simulink model "myo_sfun_one_myo_imu_emg"  (R2019a)
(part 9 of 12)

  "IW{2,1}(917,:)'" : Constant  Value=[1.233818349995047913836287989397533237934112548828125;-1.4548391149698105540011283665080554783344268798828125;-0.57922557343483427327868184875114820897579193115234375;1.505800985853002149639223716803826391696929931640625;1.3314411941759825008801954027148894965648651123046875;0.383690991252394197896791183666209690272808074951171875;-1.31641986432559665587405106634832918643951416015625;-1.081150647899540739871326877619139850139617919921875]
      mask Display: e = 0.06;c1 = [120 150 230]/255;c2 = ([120 150 230]+0)/383;c3 = ([120 150 230]+128)/383;patch([0 1 1 0],[0 0 1 1],c1);patch([0 1 1 1-e 1-e 0+e],[0 0 1 1-e 0+e 0+e],c2);patch([0 0 1 1-e 0+e 0+e],[0 1 1 1-e 1-e 0+e],c3);plot([0 1 1 0 0],[0 0 1 1 0]);disp('weights');
  "IW{2,1}(918,:)'" : Constant  Value=[0.97625063577431225869673880879417993128299713134765625;-1.796096170135296432590621407143771648406982421875;-0.93306574008488973870356630868627689778804779052734375;0.3230690155631952276138463275856338441371917724609375;-1.6813590513011014149213906421209685504436492919921875;-0.0308654014504310715560908562338227056898176670074462890625;-1.698210746333440379629564631613902747631072998046875;-0.535703429127936114895192076801322400569915771484375]
      mask Display: e = 0.06;c1 = [120 150 230]/255;c2 = ([120 150 230]+0)/383;c3 = ([120 150 230]+128)/383;patch([0 1 1 0],[0 0 1 1],c1);patch([0 1 1 1-e 1-e 0+e],[0 0 1 1-e 0+e 0+e],c2);patch([0 0 1 1-e 0+e 0+e],[0 1 1 1-e 1-e 0+e],c3);plot([0 1 1 0 0],[0 0 1 1 0]);disp('weights');
  "IW{2,1}(919,:)'" : Constant  Value=[-0.062478952272413797175421024121533264406025409698486328125;-0.96688876038711268900982531704357825219631195068359375;-1.3113773268668922344915017674793489277362823486328125;1.2445006808411676058057082627783529460430145263671875;1.8892739940812457444252459026756696403026580810546875;0.91363180064540261415828581448295153677463531494140625;1.472319784430609512781984449247829616069793701171875;0.2367699596751023649598977272034971974790096282958984375]
      mask Display: e = 0.06;c1 = [120 150 230]/255;c2 = ([120 150 230]+0)/383;c3 = ([120 150 230]+128)/383;patch([0 1 1 0],[0 0 1 1],c1);patch([0 1 1 1-e 1-e 0+e],[0 0 1 1-e 0+e 0+e],c2);patch([0 0 1 1-e 0+e 0+e],[0 1 1 1-e 1-e 0+e],c3);plot([0 1 1 0 0],[0 0 1 1 0]);disp('weights');
  "IW{2,1}(92,:)'" : Constant  Value=[1.569622482339936286876991289318539202213287353515625;-1.6722158298112417273983965060324408113956451416015625;1.3747281294294364517583062479388900101184844970703125;-0.84787514995572943465873549939715303480625152587890625;0.7901565381123225595416670330450870096683502197265625;-0.508869894851785797840193481533788144588470458984375;-0.0235341566085378005313000215892316191457211971282958984375;1.5106950540518997438965698165702633559703826904296875]
      mask Display: e = 0.06;c1 = [120 150 230]/255;c2 = ([120 150 230]+0)/383;c3 = ([120 150 230]+128)/383;patch([0 1 1 0],[0 0 1 1],c1);patch([0 1 1 1-e 1-e 0+e],[0 0 1 1-e 0+e 0+e],c2);patch([0 0 1 1-e 0+e 0+e],[0 1 1 1-e 1-e 0+e],c3);plot([0 1 1 0 0],[0 0 1 1 0]);disp('weights');
  "IW{2,1}(920,:)'" : Constant  Value=[-1.78069224270060377790514394291676580905914306640625;-1.756790645973715481176213870639912784099578857421875;0.8717506085395985149233410993474535644054412841796875;0.632232144906200499434589801239781081676483154296875;0.09756681000700063999264699532432132400572299957275390625;1.5168287045180723904280739589012227952480316162109375;0.0183378640337535682436342909795712330378592014312744140625;-1.1205682288554947856340504586114548146724700927734375]
      mask Display: e = 0.06;c1 = [120 150 230]/255;c2 = ([120 150 230]+0)/383;c3 = ([120 150 230]+128)/383;patch([0 1 1 0],[0 0 1 1],c1);patch([0 1 1 1-e 1-e 0+e],[0 0 1 1-e 0+e 0+e],c2);patch([0 0 1 1-e 0+e 0+e],[0 1 1 1-e 1-e 0+e],c3);plot([0 1 1 0 0],[0 0 1 1 0]);disp('weights');
  "IW{2,1}(921,:)'" : Constant  Value=[1.2340381365703052551907603628933429718017578125;-0.7941917179881461397172870420035906136035919189453125;0.92869565930659325747598131783888675272464752197265625;-1.48036562469159260757578522316180169582366943359375;-1.2877727848034314916958464891649782657623291015625;1.4188258803790863016303092081216163933277130126953125;1.3505426288009514390608956091455183923244476318359375;0.56256213396588250486018978335778228938579559326171875]
      mask Display: e = 0.06;c1 = [120 150 230]/255;c2 = ([120 150 230]+0)/383;c3 = ([120 150 230]+128)/383;patch([0 1 1 0],[0 0 1 1],c1);patch([0 1 1 1-e 1-e 0+e],[0 0 1 1-e 0+e 0+e],c2);patch([0 0 1 1-e 0+e 0+e],[0 1 1 1-e 1-e 0+e],c3);plot([0 1 1 0 0],[0 0 1 1 0]);disp('weights');
  "IW{2,1}(922,:)'" : Constant  Value=[0.52907092398030197699654308962635695934295654296875;-0.56376371958651005922291687966207973659038543701171875;1.962985257292654051042291030171327292919158935546875;-1.296892178749799118264718345017172396183013916015625;0.4288987352076383263721481853281147778034210205078125;-1.2792060230482646954186520815710537135601043701171875;0.00643970491984885602676502713848094572313129901885986328125;-1.7085131522321892472149329478270374238491058349609375]
      mask Display: e = 0.06;c1 = [120 150 230]/255;c2 = ([120 150 230]+0)/383;c3 = ([120 150 230]+128)/383;patch([0 1 1 0],[0 0 1 1],c1);patch([0 1 1 1-e 1-e 0+e],[0 0 1 1-e 0+e 0+e],c2);patch([0 0 1 1-e 0+e 0+e],[0 1 1 1-e 1-e 0+e],c3);plot([0 1 1 0 0],[0 0 1 1 0]);disp('weights');
  "IW{2,1}(923,:)'" : Constant  Value=[-1.4344793229196290962335069707478396594524383544921875;-1.433847325507824788104471736005507409572601318359375;0.85757048812909852930630449918680824339389801025390625;1.4320646508188261680771802275558002293109893798828125;0.7544209783935496016482602499308995902538299560546875;0.60201451337752731607366740718134678900241851806640625;-1.0747759747253453621596008815686218440532684326171875;-1.4299949869762149656793326357728801667690277099609375]
      mask Display: e = 0.06;c1 = [120 150 230]/255;c2 = ([120 150 230]+0)/383;c3 = ([120 150 230]+128)/383;patch([0 1 1 0],[0 0 1 1],c1);patch([0 1 1 1-e 1-e 0+e],[0 0 1 1-e 0+e 0+e],c2);patch([0 0 1 1-e 0+e 0+e],[0 1 1 1-e 1-e 0+e],c3);plot([0 1 1 0 0],[0 0 1 1 0]);disp('weights');
  "IW{2,1}(924,:)'" : Constant  Value=[1.46370152051110746782569549395702779293060302734375;-1.45028040887480802467734974925406277179718017578125;-1.693963962550077528845804408774711191654205322265625;-1.3273955542829203313459629498538561165332794189453125;0.2477303836859091890065798224895843304693698883056640625;0.410986296970826614494143314004759304225444793701171875;-1.34217386380958725311529633472673594951629638671875;0.334924337123925497383680749408085830509662628173828125]
      mask Display: e = 0.06;c1 = [120 150 230]/255;c2 = ([120 150 230]+0)/383;c3 = ([120 150 230]+128)/383;patch([0 1 1 0],[0 0 1 1],c1);patch([0 1 1 1-e 1-e 0+e],[0 0 1 1-e 0+e 0+e],c2);patch([0 0 1 1-e 0+e 0+e],[0 1 1 1-e 1-e 0+e],c3);plot([0 1 1 0 0],[0 0 1 1 0]);disp('weights');
  "IW{2,1}(925,:)'" : Constant  Value=[-0.80343815628262149619587262350250966846942901611328125;1.23324691550459508704307154403068125247955322265625;-0.316568060198488876455513718610745854675769805908203125;-1.945293161466664866310338766197673976421356201171875;0.5960065168583223993437059107236564159393310546875;1.6328048241174808463682666115346364676952362060546875;-1.23835047078790072561105262138880789279937744140625;-0.65057393111039230060299587421468459069728851318359375]
      mask Display: e = 0.06;c1 = [120 150 230]/255;c2 = ([120 150 230]+0)/383;c3 = ([120 150 230]+128)/383;patch([0 1 1 0],[0 0 1 1],c1);patch([0 1 1 1-e 1-e 0+e],[0 0 1 1-e 0+e 0+e],c2);patch([0 0 1 1-e 0+e 0+e],[0 1 1 1-e 1-e 0+e],c3);plot([0 1 1 0 0],[0 0 1 1 0]);disp('weights');
  "IW{2,1}(926,:)'" : Constant  Value=[0.09118175811866091606816553394310176372528076171875;-0.8389622353409638133570069840061478316783905029296875;1.210727032626933041825623149634338915348052978515625;1.293501909600718757786808055243454873561859130859375;-1.6284239784387757321582057556952349841594696044921875;-1.60098607932530256903191911987960338592529296875;-1.2636191412525807908906472221133299171924591064453125;-0.36179817522204160695764585398137569427490234375]
      mask Display: e = 0.06;c1 = [120 150 230]/255;c2 = ([120 150 230]+0)/383;c3 = ([120 150 230]+128)/383;patch([0 1 1 0],[0 0 1 1],c1);patch([0 1 1 1-e 1-e 0+e],[0 0 1 1-e 0+e 0+e],c2);patch([0 0 1 1-e 0+e 0+e],[0 1 1 1-e 1-e 0+e],c3);plot([0 1 1 0 0],[0 0 1 1 0]);disp('weights');
  "IW{2,1}(927,:)'" : Constant  Value=[-1.4683117468887691980938825508928857743740081787109375;-1.125812298427818713975057107745669782161712646484375;1.402350909702253289879081421531736850738525390625;1.17972039460394029219969525001943111419677734375;-1.189874093891304607240044788341037929058074951171875;0.82527880489423888210609447924070991575717926025390625;1.3554320717921399808147953081061132252216339111328125;0.445007997019099266200470310650416649878025054931640625]
      mask Display: e = 0.06;c1 = [120 150 230]/255;c2 = ([120 150 230]+0)/383;c3 = ([120 150 230]+128)/383;patch([0 1 1 0],[0 0 1 1],c1);patch([0 1 1 1-e 1-e 0+e],[0 0 1 1-e 0+e 0+e],c2);patch([0 0 1 1-e 0+e 0+e],[0 1 1 1-e 1-e 0+e],c3);plot([0 1 1 0 0],[0 0 1 1 0]);disp('weights');
  "IW{2,1}(928,:)'" : Constant  Value=[0.20559520258321006824786536526517011225223541259765625;0.3496458011807741517174008549773134291172027587890625;0.7578976435515378806684338997001759707927703857421875;-0.96497414503002676422482863927143625915050506591796875;-2.2761285455608035732666394324041903018951416015625;-2.114827771400021649839118254021741449832916259765625;0.5069606864833466897124480965430848300457000732421875;0.53269535080165086871062385398545302450656890869140625]
      mask Display: e = 0.06;c1 = [120 150 230]/255;c2 = ([120 150 230]+0)/383;c3 = ([120 150 230]+128)/383;patch([0 1 1 0],[0 0 1 1],c1);patch([0 1 1 1-e 1-e 0+e],[0 0 1 1-e 0+e 0+e],c2);patch([0 0 1 1-e 0+e 0+e],[0 1 1 1-e 1-e 0+e],c3);plot([0 1 1 0 0],[0 0 1 1 0]);disp('weights');
  "IW{2,1}(929,:)'" : Constant  Value=[0.83300144991458946464035761891864240169525146484375;-1.0378524650019234076836482927319593727588653564453125;-0.1574880296440317462014490956789813935756683349609375;-0.158074214384277933476141697610728442668914794921875;1.3647263842503016828544559757574461400508880615234375;1.2931349855028388962097096737124957144260406494140625;-0.040154367939153355615555796020998968742787837982177734375;2.380261894743207928826222996576689183712005615234375]
      mask Display: e = 0.06;c1 = [120 150 230]/255;c2 = ([120 150 230]+0)/383;c3 = ([120 150 230]+128)/383;patch([0 1 1 0],[0 0 1 1],c1);patch([0 1 1 1-e 1-e 0+e],[0 0 1 1-e 0+e 0+e],c2);patch([0 0 1 1-e 0+e 0+e],[0 1 1 1-e 1-e 0+e],c3);plot([0 1 1 0 0],[0 0 1 1 0]);disp('weights');
  "IW{2,1}(93,:)'" : Constant  Value=[-1.251296272410225896010160795412957668304443359375;1.501077551730921388895012569264508783817291259765625;-1.20650068227487228256222806521691381931304931640625;-1.4767900871354211478347906449926085770130157470703125;1.23206725601141098280777441686950623989105224609375;0.6159584242327740266631508347927592694759368896484375;-0.61376517944694908290870216660550795495510101318359375;1.160008933468915426345802188734523952007293701171875]
      mask Display: e = 0.06;c1 = [120 150 230]/255;c2 = ([120 150 230]+0)/383;c3 = ([120 150 230]+128)/383;patch([0 1 1 0],[0 0 1 1],c1);patch([0 1 1 1-e 1-e 0+e],[0 0 1 1-e 0+e 0+e],c2);patch([0 0 1 1-e 0+e 0+e],[0 1 1 1-e 1-e 0+e],c3);plot([0 1 1 0 0],[0 0 1 1 0]);disp('weights');
  "IW{2,1}(930,:)'" : Constant  Value=[0.459515014521598208485642089726752601563930511474609375;1.274038251996577830738033298985101282596588134765625;-0.462123489601668213655472072787233628332614898681640625;-1.2313600730026921237225678851245902478694915771484375;2.324661295404313765544657144346274435520172119140625;-1.275147702745309974403653541230596601963043212890625;0.006852607156798958508436836467581088072620332241058349609375;0.64580748349911776262644025337067432701587677001953125]
      mask Display: e = 0.06;c1 = [120 150 230]/255;c2 = ([120 150 230]+0)/383;c3 = ([120 150 230]+128)/383;patch([0 1 1 0],[0 0 1 1],c1);patch([0 1 1 1-e 1-e 0+e],[0 0 1 1-e 0+e 0+e],c2);patch([0 0 1 1-e 0+e 0+e],[0 1 1 1-e 1-e 0+e],c3);plot([0 1 1 0 0],[0 0 1 1 0]);disp('weights');
  "IW{2,1}(931,:)'" : Constant  Value=[0.1280454771649393863608423771438538096845149993896484375;0.59353344051585155138894833726226352155208587646484375;-1.2413483482938836299780405170167796313762664794921875;-1.387491740431027853475143274408765137195587158203125;-0.41476915329622709993628859592718072235584259033203125;2.049464981171696731365727828233502805233001708984375;0.94176951285771381972011795369326137006282806396484375;-1.3840451161403819480000265684793703258037567138671875]
      mask Display: e = 0.06;c1 = [120 150 230]/255;c2 = ([120 150 230]+0)/383;c3 = ([120 150 230]+128)/383;patch([0 1 1 0],[0 0 1 1],c1);patch([0 1 1 1-e 1-e 0+e],[0 0 1 1-e 0+e 0+e],c2);patch([0 0 1 1-e 0+e 0+e],[0 1 1 1-e 1-e 0+e],c3);plot([0 1 1 0 0],[0 0 1 1 0]);disp('weights');
  "IW{2,1}(932,:)'" : Constant  Value=[0.35977187717559921953380808190559037029743194580078125;1.7540295201390023738241552564431913197040557861328125;-1.43762591560315744487752454006113111972808837890625;-0.006080287386095576708522347786356476717628538608551025390625;-0.311097464246324062475679284034413285553455352783203125;-1.2697604847810930461804446167661808431148529052734375;0.94609842053890746971234193551936186850070953369140625;1.77723577742588734196260702447034418582916259765625]
      mask Display: e = 0.06;c1 = [120 150 230]/255;c2 = ([120 150 230]+0)/383;c3 = ([120 150 230]+128)/383;patch([0 1 1 0],[0 0 1 1],c1);patch([0 1 1 1-e 1-e 0+e],[0 0 1 1-e 0+e 0+e],c2);patch([0 0 1 1-e 0+e 0+e],[0 1 1 1-e 1-e 0+e],c3);plot([0 1 1 0 0],[0 0 1 1 0]);disp('weights');
  "IW{2,1}(933,:)'" : Constant  Value=[-0.55971507988235524866382775144302286207675933837890625;1.344039743685524701533040570211596786975860595703125;1.284763347918191467300630392855964601039886474609375;-1.55473640286817182953882365836761891841888427734375;-1.488883701200015341470361818210221827030181884765625;-0.14626156873139828373808768446906469762325286865234375;-0.6249568527413627005984153583995066583156585693359375;-1.4858424850743496836713575248722918331623077392578125]
      mask Display: e = 0.06;c1 = [120 150 230]/255;c2 = ([120 150 230]+0)/383;c3 = ([120 150 230]+128)/383;patch([0 1 1 0],[0 0 1 1],c1);patch([0 1 1 1-e 1-e 0+e],[0 0 1 1-e 0+e 0+e],c2);patch([0 0 1 1-e 0+e 0+e],[0 1 1 1-e 1-e 0+e],c3);plot([0 1 1 0 0],[0 0 1 1 0]);disp('weights');
  "IW{2,1}(934,:)'" : Constant  Value=[-1.752013618542566320002151769585907459259033203125;1.3291169268141735937405201184446923434734344482421875;-0.6787032919514575102226672242977656424045562744140625;0.490359468964445321947920319871627725660800933837890625;-1.57210680514284195652408016030676662921905517578125;-0.01000360648531075681566537838307340280152857303619384765625;-0.285459327197532142239566610442125238478183746337890625;-1.7110715408113696955894056372926570475101470947265625]
      mask Display: e = 0.06;c1 = [120 150 230]/255;c2 = ([120 150 230]+0)/383;c3 = ([120 150 230]+128)/383;patch([0 1 1 0],[0 0 1 1],c1);patch([0 1 1 1-e 1-e 0+e],[0 0 1 1-e 0+e 0+e],c2);patch([0 0 1 1-e 0+e 0+e],[0 1 1 1-e 1-e 0+e],c3);plot([0 1 1 0 0],[0 0 1 1 0]);disp('weights');
  "IW{2,1}(935,:)'" : Constant  Value=[-1.6614565255023199252804033676511608064174652099609375;0.734584289137682588943789596669375896453857421875;1.0579080812622836393899206086643971502780914306640625;0.52610990226821907622678509142133407294750213623046875;1.34837736401491969928656544652767479419708251953125;1.0300380949842151689921365687041543424129486083984375;-0.87449305309208369418882966783712618052959442138671875;1.5773892164364966550493818431277759373188018798828125]
      mask Display: e = 0.06;c1 = [120 150 230]/255;c2 = ([120 150 230]+0)/383;c3 = ([120 150 230]+128)/383;patch([0 1 1 0],[0 0 1 1],c1);patch([0 1 1 1-e 1-e 0+e],[0 0 1 1-e 0+e 0+e],c2);patch([0 0 1 1-e 0+e 0+e],[0 1 1 1-e 1-e 0+e],c3);plot([0 1 1 0 0],[0 0 1 1 0]);disp('weights');
  "IW{2,1}(936,:)'" : Constant  Value=[0.022714479700087643332384601535522961057722568511962890625;-1.573558474179254318414677982218563556671142578125;1.3066200625597179652004342642612755298614501953125;-0.1673441857289472423087062225022236816585063934326171875;1.8960528148548283500218758490518666803836822509765625;1.340663180394818798646383584127761423587799072265625;0.55978272292861486203463527999701909720897674560546875;1.049900791636255714678327422006987035274505615234375]
      mask Display: e = 0.06;c1 = [120 150 230]/255;c2 = ([120 150 230]+0)/383;c3 = ([120 150 230]+128)/383;patch([0 1 1 0],[0 0 1 1],c1);patch([0 1 1 1-e 1-e 0+e],[0 0 1 1-e 0+e 0+e],c2);patch([0 0 1 1-e 0+e 0+e],[0 1 1 1-e 1-e 0+e],c3);plot([0 1 1 0 0],[0 0 1 1 0]);disp('weights');
  "IW{2,1}(937,:)'" : Constant  Value=[0.829643574270976902340635206201113760471343994140625;2.22733223083989262391924057737924158573150634765625;-0.79551413202837040206105712059070356190204620361328125;0.9418309463257037439376517795608378946781158447265625;-0.774473438339178255063188771600835025310516357421875;1.300848255993976909650200468604452908039093017578125;1.2493782215186015616126269378582946956157684326171875;0.021557995414638909947857570159612805582582950592041015625]
      mask Display: e = 0.06;c1 = [120 150 230]/255;c2 = ([120 150 230]+0)/383;c3 = ([120 150 230]+128)/383;patch([0 1 1 0],[0 0 1 1],c1);patch([0 1 1 1-e 1-e 0+e],[0 0 1 1-e 0+e 0+e],c2);patch([0 0 1 1-e 0+e 0+e],[0 1 1 1-e 1-e 0+e],c3);plot([0 1 1 0 0],[0 0 1 1 0]);disp('weights');
  "IW{2,1}(938,:)'" : Constant  Value=[1.345901355534946386427463949075900018215179443359375;-2.02660768801359747470769434585236012935638427734375;1.352468657955171682516493092407472431659698486328125;-1.3978356390675228393405404858640395104885101318359375;-0.9061008277153874690412749259849078953266143798828125;-0.0980897452544215731062848817600752227008342742919921875;0.72250261894200551449074509946512989699840545654296875;-0.209980731838069145656078262618393637239933013916015625]
      mask Display: e = 0.06;c1 = [120 150 230]/255;c2 = ([120 150 230]+0)/383;c3 = ([120 150 230]+128)/383;patch([0 1 1 0],[0 0 1 1],c1);patch([0 1 1 1-e 1-e 0+e],[0 0 1 1-e 0+e 0+e],c2);patch([0 0 1 1-e 0+e 0+e],[0 1 1 1-e 1-e 0+e],c3);plot([0 1 1 0 0],[0 0 1 1 0]);disp('weights');
  "IW{2,1}(939,:)'" : Constant  Value=[-0.82112012880838258777060900683864019811153411865234375;-1.930845595022031790932715011877007782459259033203125;-1.15556707295993010831125502591021358966827392578125;1.179015320370934372107285525999031960964202880859375;-1.3288541314620074818009243244887329638004302978515625;1.2953923768230557467262542559183202683925628662109375;-0.2042937924653980275024878210388123989105224609375;-0.6321215672831559384547972513246349990367889404296875]
      mask Display: e = 0.06;c1 = [120 150 230]/255;c2 = ([120 150 230]+0)/383;c3 = ([120 150 230]+128)/383;patch([0 1 1 0],[0 0 1 1],c1);patch([0 1 1 1-e 1-e 0+e],[0 0 1 1-e 0+e 0+e],c2);patch([0 0 1 1-e 0+e 0+e],[0 1 1 1-e 1-e 0+e],c3);plot([0 1 1 0 0],[0 0 1 1 0]);disp('weights');
  "IW{2,1}(94,:)'" : Constant  Value=[-0.89691044877446557403999349844525568187236785888671875;-1.9703867433167996381371267489157617092132568359375;-1.2689724396955994745184170824359171092510223388671875;-1.102188217761382649229062735685147345066070556640625;0.212948896185985281359620557850576005876064300537109375;1.4063245905018693093779802438803017139434814453125;0.5220856679645944353751474409364163875579833984375;1.2669379614301450320823505535372532904148101806640625]
      mask Display: e = 0.06;c1 = [120 150 230]/255;c2 = ([120 150 230]+0)/383;c3 = ([120 150 230]+128)/383;patch([0 1 1 0],[0 0 1 1],c1);patch([0 1 1 1-e 1-e 0+e],[0 0 1 1-e 0+e 0+e],c2);patch([0 0 1 1-e 0+e 0+e],[0 1 1 1-e 1-e 0+e],c3);plot([0 1 1 0 0],[0 0 1 1 0]);disp('weights');
  "IW{2,1}(940,:)'" : Constant  Value=[-1.9284641361261212200162162844208069145679473876953125;-0.6923000284259206438264300231821835041046142578125;-0.01547752074768899387124942990112685947678983211517333984375;-1.51835172518999694801777877728454768657684326171875;1.1196957434104588546830427731038071215152740478515625;-0.54044636995000117085652391324401833117008209228515625;-0.40395263561673733221368820522911846637725830078125;-1.6755700378273326034417323171510361135005950927734375]
      mask Display: e = 0.06;c1 = [120 150 230]/255;c2 = ([120 150 230]+0)/383;c3 = ([120 150 230]+128)/383;patch([0 1 1 0],[0 0 1 1],c1);patch([0 1 1 1-e 1-e 0+e],[0 0 1 1-e 0+e 0+e],c2);patch([0 0 1 1-e 0+e 0+e],[0 1 1 1-e 1-e 0+e],c3);plot([0 1 1 0 0],[0 0 1 1 0]);disp('weights');
  "IW{2,1}(941,:)'" : Constant  Value=[-0.67344134392942589517616625016671605408191680908203125;-1.7808742618691166814670623352867551147937774658203125;1.4264091809267844812580960933701135218143463134765625;1.911975433919925304593334658420644700527191162109375;-0.7236950162813198250688628831994719803333282470703125;-0.370798693591568639948974350772914476692676544189453125;-0.329395901859115713961045912583358585834503173828125;-0.96579283248583458476588248231564648449420928955078125]
      mask Display: e = 0.06;c1 = [120 150 230]/255;c2 = ([120 150 230]+0)/383;c3 = ([120 150 230]+128)/383;patch([0 1 1 0],[0 0 1 1],c1);patch([0 1 1 1-e 1-e 0+e],[0 0 1 1-e 0+e 0+e],c2);patch([0 0 1 1-e 0+e 0+e],[0 1 1 1-e 1-e 0+e],c3);plot([0 1 1 0 0],[0 0 1 1 0]);disp('weights');
  "IW{2,1}(942,:)'" : Constant  Value=[-1.64674280850280663202056530280970036983489990234375;-1.5001296336770109096647729529649950563907623291015625;0.08935031672762583365710042926366440951824188232421875;-0.921153845618884137280701907002367079257965087890625;-0.483100667039175146744156563727301545441150665283203125;-0.7427427715172323363646000871085561811923980712890625;-1.6797167079109793785818283140542916953563690185546875;-1.26337657129443758918796447687782347202301025390625]
      mask Display: e = 0.06;c1 = [120 150 230]/255;c2 = ([120 150 230]+0)/383;c3 = ([120 150 230]+128)/383;patch([0 1 1 0],[0 0 1 1],c1);patch([0 1 1 1-e 1-e 0+e],[0 0 1 1-e 0+e 0+e],c2);patch([0 0 1 1-e 0+e 0+e],[0 1 1 1-e 1-e 0+e],c3);plot([0 1 1 0 0],[0 0 1 1 0]);disp('weights');
  "IW{2,1}(943,:)'" : Constant  Value=[-0.6229731159529052764156631383229978382587432861328125;0.98169370896949093019401288984226994216442108154296875;-1.6364243634393706994245576424873434007167816162109375;0.950796335976273443435502485954202711582183837890625;1.0949390867111337133366077978280372917652130126953125;1.515828966336887351218365438398905098438262939453125;0.9413789297321477622659813278005458414554595947265625;-1.229582187669542303609659938956610858440399169921875]
      mask Display: e = 0.06;c1 = [120 150 230]/255;c2 = ([120 150 230]+0)/383;c3 = ([120 150 230]+128)/383;patch([0 1 1 0],[0 0 1 1],c1);patch([0 1 1 1-e 1-e 0+e],[0 0 1 1-e 0+e 0+e],c2);patch([0 0 1 1-e 0+e 0+e],[0 1 1 1-e 1-e 0+e],c3);plot([0 1 1 0 0],[0 0 1 1 0]);disp('weights');
  "IW{2,1}(944,:)'" : Constant  Value=[1.6916018903944003426431663683615624904632568359375;1.630736797217114286695505143143236637115478515625;1.2800499861010774527159128410858102142810821533203125;0.94571459497293342000290294890874065458774566650390625;0.3303592853984034238834510688320733606815338134765625;-1.4924581285519600282185592732275836169719696044921875;-0.79231501501053436253840800418402068316936492919921875;-0.03770714380415697564163934885073103941977024078369140625]
      mask Display: e = 0.06;c1 = [120 150 230]/255;c2 = ([120 150 230]+0)/383;c3 = ([120 150 230]+128)/383;patch([0 1 1 0],[0 0 1 1],c1);patch([0 1 1 1-e 1-e 0+e],[0 0 1 1-e 0+e 0+e],c2);patch([0 0 1 1-e 0+e 0+e],[0 1 1 1-e 1-e 0+e],c3);plot([0 1 1 0 0],[0 0 1 1 0]);disp('weights');
  "IW{2,1}(945,:)'" : Constant  Value=[-0.07490041787247413151984432033714256249368190765380859375;-0.2172170720689318990093141792385722510516643524169921875;0.75781279649731825287517494871281087398529052734375;1.821447104661903182432070025242865085601806640625;-0.7881694043895723922332763322629034519195556640625;-1.684895341352864672757050357176922261714935302734375;-0.2646422506319991985179740368039347231388092041015625;-1.8832174078616155110665886240894906222820281982421875]
      mask Display: e = 0.06;c1 = [120 150 230]/255;c2 = ([120 150 230]+0)/383;c3 = ([120 150 230]+128)/383;patch([0 1 1 0],[0 0 1 1],c1);patch([0 1 1 1-e 1-e 0+e],[0 0 1 1-e 0+e 0+e],c2);patch([0 0 1 1-e 0+e 0+e],[0 1 1 1-e 1-e 0+e],c3);plot([0 1 1 0 0],[0 0 1 1 0]);disp('weights');
  "IW{2,1}(946,:)'" : Constant  Value=[-1.61656003434635398008367701550014317035675048828125;-1.5618385803786349885768913736683316528797149658203125;-0.277455301741910964619108881379361264407634735107421875;1.3992954332120628446745058681699447333812713623046875;-1.3023534400012752865194443074869923293590545654296875;0.9148572075036749406962144348653964698314666748046875;0.247215396692398059474982119354535825550556182861328125;-1.1568899404959995802499861383694224059581756591796875]
      mask Display: e = 0.06;c1 = [120 150 230]/255;c2 = ([120 150 230]+0)/383;c3 = ([120 150 230]+128)/383;patch([0 1 1 0],[0 0 1 1],c1);patch([0 1 1 1-e 1-e 0+e],[0 0 1 1-e 0+e 0+e],c2);patch([0 0 1 1-e 0+e 0+e],[0 1 1 1-e 1-e 0+e],c3);plot([0 1 1 0 0],[0 0 1 1 0]);disp('weights');
  "IW{2,1}(947,:)'" : Constant  Value=[0.67278616972188653999609186939778737723827362060546875;0.315790583508263000833693467939156107604503631591796875;-1.9304221908873084867508396200719289481639862060546875;1.46464184402568076137640673550777137279510498046875;0.324555519664747660346648672202718444168567657470703125;1.8096189180068671387147105633630417287349700927734375;-0.297396691982909022744507865354535169899463653564453125;-1.06090862285816722732079142588190734386444091796875]
      mask Display: e = 0.06;c1 = [120 150 230]/255;c2 = ([120 150 230]+0)/383;c3 = ([120 150 230]+128)/383;patch([0 1 1 0],[0 0 1 1],c1);patch([0 1 1 1-e 1-e 0+e],[0 0 1 1-e 0+e 0+e],c2);patch([0 0 1 1-e 0+e 0+e],[0 1 1 1-e 1-e 0+e],c3);plot([0 1 1 0 0],[0 0 1 1 0]);disp('weights');
  "IW{2,1}(948,:)'" : Constant  Value=[0.69274726211865711444914950334350578486919403076171875;1.75931371522753021707785592298023402690887451171875;-0.334146673453465548053742395495646633207798004150390625;1.416235474757840062665081859449855983257293701171875;-1.49001771332762444899344700388610363006591796875;-0.4963658635882872705025192772154696285724639892578125;1.6882243163268089158890461476403288543224334716796875;-0.106785619132828191180095700474339537322521209716796875]
      mask Display: e = 0.06;c1 = [120 150 230]/255;c2 = ([120 150 230]+0)/383;c3 = ([120 150 230]+128)/383;patch([0 1 1 0],[0 0 1 1],c1);patch([0 1 1 1-e 1-e 0+e],[0 0 1 1-e 0+e 0+e],c2);patch([0 0 1 1-e 0+e 0+e],[0 1 1 1-e 1-e 0+e],c3);plot([0 1 1 0 0],[0 0 1 1 0]);disp('weights');
  "IW{2,1}(949,:)'" : Constant  Value=[0.26027926239215359860423859572620131075382232666015625;0.55307858353162020481619265410699881613254547119140625;1.051142655215786536615496515878476202487945556640625;-1.3810340222430579348866785949212498962879180908203125;1.3515319635994840208326195352128706872463226318359375;1.838861764011227695192474129726178944110870361328125;-1.0853865001339315643491545415599830448627471923828125;1.115992553842682699638544363551773130893707275390625]
      mask Display: e = 0.06;c1 = [120 150 230]/255;c2 = ([120 150 230]+0)/383;c3 = ([120 150 230]+128)/383;patch([0 1 1 0],[0 0 1 1],c1);patch([0 1 1 1-e 1-e 0+e],[0 0 1 1-e 0+e 0+e],c2);patch([0 0 1 1-e 0+e 0+e],[0 1 1 1-e 1-e 0+e],c3);plot([0 1 1 0 0],[0 0 1 1 0]);disp('weights');
  "IW{2,1}(95,:)'" : Constant  Value=[0.005290517661980498852203336213051443337462842464447021484375;-1.6497505516666877145581793229212053120136260986328125;1.620443822731480576493368062074296176433563232421875;0.16986718877335504895853546258877031505107879638671875;1.054192073111287708542249674792401492595672607421875;2.0288246145218096216922276653349399566650390625;0.76925751328801295070292098898789845407009124755859375;0.305950453478517570005124071030877530574798583984375]
      mask Display: e = 0.06;c1 = [120 150 230]/255;c2 = ([120 150 230]+0)/383;c3 = ([120 150 230]+128)/383;patch([0 1 1 0],[0 0 1 1],c1);patch([0 1 1 1-e 1-e 0+e],[0 0 1 1-e 0+e 0+e],c2);patch([0 0 1 1-e 0+e 0+e],[0 1 1 1-e 1-e 0+e],c3);plot([0 1 1 0 0],[0 0 1 1 0]);disp('weights');
  "IW{2,1}(950,:)'" : Constant  Value=[0.2118013824636972020076797207366325892508029937744140625;0.0222517894993314417628749168898139032535254955291748046875;-0.59674814348700089272625746161793358623981475830078125;0.11734950071789367054275743385005625896155834197998046875;-1.024961618939134400108059708145447075366973876953125;1.9878634122041984877427012179396115243434906005859375;0.2500324382013621171694239819771610200405120849609375;2.353073982785186313293479543062858283519744873046875]
      mask Display: e = 0.06;c1 = [120 150 230]/255;c2 = ([120 150 230]+0)/383;c3 = ([120 150 230]+128)/383;patch([0 1 1 0],[0 0 1 1],c1);patch([0 1 1 1-e 1-e 0+e],[0 0 1 1-e 0+e 0+e],c2);patch([0 0 1 1-e 0+e 0+e],[0 1 1 1-e 1-e 0+e],c3);plot([0 1 1 0 0],[0 0 1 1 0]);disp('weights');
  "IW{2,1}(951,:)'" : Constant  Value=[-0.80119265775817571917372106327093206346035003662109375;0.29490648552127052273164053985965438187122344970703125;1.9174919947240212092509636931936256587505340576171875;2.132198923601664741767081068246625363826751708984375;0.60462532016717485117140995498630218207836151123046875;0.819228102816961012422325438819825649261474609375;-1.0039939427206672206693838234059512615203857421875;0.252263222953873877951735948954592458903789520263671875]
      mask Display: e = 0.06;c1 = [120 150 230]/255;c2 = ([120 150 230]+0)/383;c3 = ([120 150 230]+128)/383;patch([0 1 1 0],[0 0 1 1],c1);patch([0 1 1 1-e 1-e 0+e],[0 0 1 1-e 0+e 0+e],c2);patch([0 0 1 1-e 0+e 0+e],[0 1 1 1-e 1-e 0+e],c3);plot([0 1 1 0 0],[0 0 1 1 0]);disp('weights');
  "IW{2,1}(952,:)'" : Constant  Value=[-1.11396737416281599308831573580391705036163330078125;-1.3865399781131342304973941281787119805812835693359375;-0.40695912110590881649585526247392408549785614013671875;1.5312662831779870753479144696029834449291229248046875;-1.49056243641590224768833650159649550914764404296875;-0.97778759670928161451541882343008182942867279052734375;1.459003140404683929176599122001789510250091552734375;0.1557717566069929671090932288279873318970203399658203125]
      mask Display: e = 0.06;c1 = [120 150 230]/255;c2 = ([120 150 230]+0)/383;c3 = ([120 150 230]+128)/383;patch([0 1 1 0],[0 0 1 1],c1);patch([0 1 1 1-e 1-e 0+e],[0 0 1 1-e 0+e 0+e],c2);patch([0 0 1 1-e 0+e 0+e],[0 1 1 1-e 1-e 0+e],c3);plot([0 1 1 0 0],[0 0 1 1 0]);disp('weights');
  "IW{2,1}(953,:)'" : Constant  Value=[0.258251700948573026384025297375046648085117340087890625;-0.67611337492076251098893635571585036814212799072265625;-1.603811521270914308701094341813586652278900146484375;-0.5681734588386808670890104622230865061283111572265625;1.8536189902244133431707950876443646848201751708984375;-1.97368043547795668501976251718588173389434814453125;-0.5127002050856710457793496971135027706623077392578125;-0.414385209771393092648139599987189285457134246826171875]
      mask Display: e = 0.06;c1 = [120 150 230]/255;c2 = ([120 150 230]+0)/383;c3 = ([120 150 230]+128)/383;patch([0 1 1 0],[0 0 1 1],c1);patch([0 1 1 1-e 1-e 0+e],[0 0 1 1-e 0+e 0+e],c2);patch([0 0 1 1-e 0+e 0+e],[0 1 1 1-e 1-e 0+e],c3);plot([0 1 1 0 0],[0 0 1 1 0]);disp('weights');
  "IW{2,1}(954,:)'" : Constant  Value=[-0.0714688518537866246393974734019138850271701812744140625;0.18673843709045756522613146444200538098812103271484375;-0.9915786198777654103508893967955373227596282958984375;-1.5692759919708876292787635975400917232036590576171875;1.3352769605693486365538547033793292939662933349609375;1.4898625418610567106014741511899046599864959716796875;1.77523436073847307170581188984215259552001953125;-0.30240620026603981518320551913348026573657989501953125]
      mask Display: e = 0.06;c1 = [120 150 230]/255;c2 = ([120 150 230]+0)/383;c3 = ([120 150 230]+128)/383;patch([0 1 1 0],[0 0 1 1],c1);patch([0 1 1 1-e 1-e 0+e],[0 0 1 1-e 0+e 0+e],c2);patch([0 0 1 1-e 0+e 0+e],[0 1 1 1-e 1-e 0+e],c3);plot([0 1 1 0 0],[0 0 1 1 0]);disp('weights');
  "IW{2,1}(955,:)'" : Constant  Value=[-1.0269687330708421324487744641373865306377410888671875;-1.0798366757184023612126111402176320552825927734375;-0.69043258483427205618454536306671798229217529296875;-0.1303232596325844816487204980148817412555217742919921875;-1.93219267415173590052290819585323333740234375;-1.670762241355885802107650306425057351589202880859375;-1.102255017013542559567440548562444746494293212890625;-0.7532878530168323205629121730453334748744964599609375]
      mask Display: e = 0.06;c1 = [120 150 230]/255;c2 = ([120 150 230]+0)/383;c3 = ([120 150 230]+128)/383;patch([0 1 1 0],[0 0 1 1],c1);patch([0 1 1 1-e 1-e 0+e],[0 0 1 1-e 0+e 0+e],c2);patch([0 0 1 1-e 0+e 0+e],[0 1 1 1-e 1-e 0+e],c3);plot([0 1 1 0 0],[0 0 1 1 0]);disp('weights');
  "IW{2,1}(956,:)'" : Constant  Value=[-1.259572927524434504675809876061975955963134765625;-1.566076891330097087262629429460503160953521728515625;0.5545948087603991272231951370486058294773101806640625;0.1225122593770910928157036323682405054569244384765625;1.5461328722284743975023957318626344203948974609375;0.430893954704071102668194725993089377880096435546875;1.07278993219239726641944798757322132587432861328125;1.686995832673343187479986227117478847503662109375]
      mask Display: e = 0.06;c1 = [120 150 230]/255;c2 = ([120 150 230]+0)/383;c3 = ([120 150 230]+128)/383;patch([0 1 1 0],[0 0 1 1],c1);patch([0 1 1 1-e 1-e 0+e],[0 0 1 1-e 0+e 0+e],c2);patch([0 0 1 1-e 0+e 0+e],[0 1 1 1-e 1-e 0+e],c3);plot([0 1 1 0 0],[0 0 1 1 0]);disp('weights');
  "IW{2,1}(957,:)'" : Constant  Value=[-1.6434029746463443277804117315099574625492095947265625;-1.258336057601832091989990658476017415523529052734375;0.32737454433715351687084194054477848112583160400390625;0.21120936373135401620260154231800697743892669677734375;-1.6819519333793599979998134585912339389324188232421875;-1.06440638730531755840047480887733399868011474609375;0.50280680651173259576580676366575062274932861328125;-1.5427191834726186048243334880680777132511138916015625]
      mask Display: e = 0.06;c1 = [120 150 230]/255;c2 = ([120 150 230]+0)/383;c3 = ([120 150 230]+128)/383;patch([0 1 1 0],[0 0 1 1],c1);patch([0 1 1 1-e 1-e 0+e],[0 0 1 1-e 0+e 0+e],c2);patch([0 0 1 1-e 0+e 0+e],[0 1 1 1-e 1-e 0+e],c3);plot([0 1 1 0 0],[0 0 1 1 0]);disp('weights');
  "IW{2,1}(958,:)'" : Constant  Value=[-1.018853361224475673196820935118012130260467529296875;1.5101623645667776596468456773436628282070159912109375;0.0034242034255393982190851520641672323108650743961334228515625;1.003591846723276059805129989399574697017669677734375;-1.3858942870144372871976656824699603021144866943359375;1.352687542195119885235499168629758059978485107421875;0.56728160579548958519779944253969006240367889404296875;-1.5707517726856281559122407998074777424335479736328125]
      mask Display: e = 0.06;c1 = [120 150 230]/255;c2 = ([120 150 230]+0)/383;c3 = ([120 150 230]+128)/383;patch([0 1 1 0],[0 0 1 1],c1);patch([0 1 1 1-e 1-e 0+e],[0 0 1 1-e 0+e 0+e],c2);patch([0 0 1 1-e 0+e 0+e],[0 1 1 1-e 1-e 0+e],c3);plot([0 1 1 0 0],[0 0 1 1 0]);disp('weights');
  "IW{2,1}(959,:)'" : Constant  Value=[-0.4406574185669251964014847544603981077671051025390625;-0.410715019488304522443655741881229914724826812744140625;-0.352068226104441439616721254424192011356353759765625;2.059402664510679326070885508670471608638763427734375;-1.0409958090927695639749117617611773312091827392578125;-1.9913627487155471929014538545743562281131744384765625;1.0051965317904218988331876971642486751079559326171875;0.483540956058685134077990142031922005116939544677734375]
      mask Display: e = 0.06;c1 = [120 150 230]/255;c2 = ([120 150 230]+0)/383;c3 = ([120 150 230]+128)/383;patch([0 1 1 0],[0 0 1 1],c1);patch([0 1 1 1-e 1-e 0+e],[0 0 1 1-e 0+e 0+e],c2);patch([0 0 1 1-e 0+e 0+e],[0 1 1 1-e 1-e 0+e],c3);plot([0 1 1 0 0],[0 0 1 1 0]);disp('weights');
  "IW{2,1}(96,:)'" : Constant  Value=[0.419246405757374318579167038478772155940532684326171875;-0.0669779989953708521088771021823049522936344146728515625;0.2115422854113650774632304774058866314589977264404296875;-0.50782976396093115756258384863031096756458282470703125;0.357548328626089928494735659114667214453220367431640625;-2.07244956583548312067932783975265920162200927734375;1.2521473769663895581061296979896724224090576171875;2.143314189418450865787235670723021030426025390625]
      mask Display: e = 0.06;c1 = [120 150 230]/255;c2 = ([120 150 230]+0)/383;c3 = ([120 150 230]+128)/383;patch([0 1 1 0],[0 0 1 1],c1);patch([0 1 1 1-e 1-e 0+e],[0 0 1 1-e 0+e 0+e],c2);patch([0 0 1 1-e 0+e 0+e],[0 1 1 1-e 1-e 0+e],c3);plot([0 1 1 0 0],[0 0 1 1 0]);disp('weights');
  "IW{2,1}(960,:)'" : Constant  Value=[-1.81324983605770650996191761805675923824310302734375;-0.86059273145285730688414105316041968762874603271484375;-1.5664151264027308396720172822824679315090179443359375;0.6894845367303157335214791601174511015415191650390625;-0.90394343784677833042451311484910547733306884765625;1.674573303986999661674417438916862010955810546875;-0.03819924795413538742838710504656773991882801055908203125;-0.67145149253797120625364414081559516489505767822265625]
      mask Display: e = 0.06;c1 = [120 150 230]/255;c2 = ([120 150 230]+0)/383;c3 = ([120 150 230]+128)/383;patch([0 1 1 0],[0 0 1 1],c1);patch([0 1 1 1-e 1-e 0+e],[0 0 1 1-e 0+e 0+e],c2);patch([0 0 1 1-e 0+e 0+e],[0 1 1 1-e 1-e 0+e],c3);plot([0 1 1 0 0],[0 0 1 1 0]);disp('weights');
  "IW{2,1}(961,:)'" : Constant  Value=[-1.6499472074669248033984558787778951227664947509765625;1.20088922343484227894805371761322021484375;1.6447708323128329421791704589850269258022308349609375;-0.887981481501101566067291059880517423152923583984375;-1.32520180444815327547303240862675011157989501953125;-0.131179755098887740327739948043017648160457611083984375;-1.1397402785706838290735731789027340710163116455078125;-0.53280778219899904701861714784172363579273223876953125]
      mask Display: e = 0.06;c1 = [120 150 230]/255;c2 = ([120 150 230]+0)/383;c3 = ([120 150 230]+128)/383;patch([0 1 1 0],[0 0 1 1],c1);patch([0 1 1 1-e 1-e 0+e],[0 0 1 1-e 0+e 0+e],c2);patch([0 0 1 1-e 0+e 0+e],[0 1 1 1-e 1-e 0+e],c3);plot([0 1 1 0 0],[0 0 1 1 0]);disp('weights');
  "IW{2,1}(962,:)'" : Constant  Value=[1.3573502858950325933307112791226245462894439697265625;-0.60731931381688120108464090662891976535320281982421875;-0.9915428741844867221999493267503567039966583251953125;-0.6027902804183693508122132698190398514270782470703125;1.21520180736901917128989225602708756923675537109375;1.7822585337978369413036716650822199881076812744140625;-1.3940052492122012584019330461160279810428619384765625;0.92264286900278580372258829811471514403820037841796875]
      mask Display: e = 0.06;c1 = [120 150 230]/255;c2 = ([120 150 230]+0)/383;c3 = ([120 150 230]+128)/383;patch([0 1 1 0],[0 0 1 1],c1);patch([0 1 1 1-e 1-e 0+e],[0 0 1 1-e 0+e 0+e],c2);patch([0 0 1 1-e 0+e 0+e],[0 1 1 1-e 1-e 0+e],c3);plot([0 1 1 0 0],[0 0 1 1 0]);disp('weights');
  "IW{2,1}(963,:)'" : Constant  Value=[-1.3167515343209206246655185168492607772350311279296875;0.559447537193499488950010345433838665485382080078125;1.58878585735060706696231136447750031948089599609375;-1.084077987127869846517569385468959808349609375;1.3597972826871316254226940145599655807018280029296875;1.3239510796163400652147856817464344203472137451171875;0.33854164740429093516382863526814617216587066650390625;-1.2540834160199099134302969105192460119724273681640625]
      mask Display: e = 0.06;c1 = [120 150 230]/255;c2 = ([120 150 230]+0)/383;c3 = ([120 150 230]+128)/383;patch([0 1 1 0],[0 0 1 1],c1);patch([0 1 1 1-e 1-e 0+e],[0 0 1 1-e 0+e 0+e],c2);patch([0 0 1 1-e 0+e 0+e],[0 1 1 1-e 1-e 0+e],c3);plot([0 1 1 0 0],[0 0 1 1 0]);disp('weights');
  "IW{2,1}(964,:)'" : Constant  Value=[-0.57177830755232317283542897712322883307933807373046875;-1.318361845342495453081710365950129926204681396484375;1.870459391293952222667940077371895313262939453125;-0.68232707282902127499113476005732081830501556396484375;0.7235961289153090003622992298915050923824310302734375;1.750578552359428829987564313341863453388214111328125;-0.1652255780773015103601863984295050613582134246826171875;1.258385077028660870013254680088721215724945068359375]
      mask Display: e = 0.06;c1 = [120 150 230]/255;c2 = ([120 150 230]+0)/383;c3 = ([120 150 230]+128)/383;patch([0 1 1 0],[0 0 1 1],c1);patch([0 1 1 1-e 1-e 0+e],[0 0 1 1-e 0+e 0+e],c2);patch([0 0 1 1-e 0+e 0+e],[0 1 1 1-e 1-e 0+e],c3);plot([0 1 1 0 0],[0 0 1 1 0]);disp('weights');
  "IW{2,1}(965,:)'" : Constant  Value=[0.2027375397307764892662618194663082249462604522705078125;-1.4414906217828209467057831716374494135379791259765625;2.09300058743209493883341565378941595554351806640625;-0.9840330538930153192467287226463668048381805419921875;-0.36414377230271366414626754703931510448455810546875;1.7068061614343454923670151401893235743045806884765625;0.60865202424146114257297313088201917707920074462890625;-0.37423839205274067598594456285354681313037872314453125]
      mask Display: e = 0.06;c1 = [120 150 230]/255;c2 = ([120 150 230]+0)/383;c3 = ([120 150 230]+128)/383;patch([0 1 1 0],[0 0 1 1],c1);patch([0 1 1 1-e 1-e 0+e],[0 0 1 1-e 0+e 0+e],c2);patch([0 0 1 1-e 0+e 0+e],[0 1 1 1-e 1-e 0+e],c3);plot([0 1 1 0 0],[0 0 1 1 0]);disp('weights');
  "IW{2,1}(966,:)'" : Constant  Value=[1.0967828584218539678118986557819880545139312744140625;-1.37792418342228284444672681274823844432830810546875;-1.1569365941362905747524791877367533743381500244140625;0.96526882643368150382912062923423945903778076171875;-0.98921332333476197362642778898589313030242919921875;1.0733257059218959117430358674027957022190093994140625;-1.274063322637671635817468995810486376285552978515625;1.437302737259740670339169810176827013492584228515625]
      mask Display: e = 0.06;c1 = [120 150 230]/255;c2 = ([120 150 230]+0)/383;c3 = ([120 150 230]+128)/383;patch([0 1 1 0],[0 0 1 1],c1);patch([0 1 1 1-e 1-e 0+e],[0 0 1 1-e 0+e 0+e],c2);patch([0 0 1 1-e 0+e 0+e],[0 1 1 1-e 1-e 0+e],c3);plot([0 1 1 0 0],[0 0 1 1 0]);disp('weights');
  "IW{2,1}(967,:)'" : Constant  Value=[-1.70776985973894124271055261488072574138641357421875;0.27690829961250484902990365299046970903873443603515625;-0.57821903266416629918467151583172380924224853515625;2.010419511329596620186066502355970442295074462890625;0.4072009625781027875035533725167624652385711669921875;-1.0905117285316012765150617269682697951793670654296875;0.27243534771448241205149543020525015890598297119140625;1.4923498116324351858708041618228890001773834228515625]
      mask Display: e = 0.06;c1 = [120 150 230]/255;c2 = ([120 150 230]+0)/383;c3 = ([120 150 230]+128)/383;patch([0 1 1 0],[0 0 1 1],c1);patch([0 1 1 1-e 1-e 0+e],[0 0 1 1-e 0+e 0+e],c2);patch([0 0 1 1-e 0+e 0+e],[0 1 1 1-e 1-e 0+e],c3);plot([0 1 1 0 0],[0 0 1 1 0]);disp('weights');
  "IW{2,1}(968,:)'" : Constant  Value=[-1.892253481005562232297734226449392735958099365234375;1.66631379754854069830116714001633226871490478515625;1.86251966480007435933430315344594419002532958984375;-0.691714216478680032906822816585190594196319580078125;-0.5969475167732294362821221511694602668285369873046875;0.2784678193456977535191754213883541524410247802734375;-0.27618477902162286152787373794126324355602264404296875;0.50343483410970468749923156792647205293178558349609375]
      mask Display: e = 0.06;c1 = [120 150 230]/255;c2 = ([120 150 230]+0)/383;c3 = ([120 150 230]+128)/383;patch([0 1 1 0],[0 0 1 1],c1);patch([0 1 1 1-e 1-e 0+e],[0 0 1 1-e 0+e 0+e],c2);patch([0 0 1 1-e 0+e 0+e],[0 1 1 1-e 1-e 0+e],c3);plot([0 1 1 0 0],[0 0 1 1 0]);disp('weights');
  "IW{2,1}(969,:)'" : Constant  Value=[-1.3147941798246802758143303435645066201686859130859375;2.309790621604359106555648395442403852939605712890625;1.4604059292313966711418515842524357140064239501953125;0.754982777773998581238856786512769758701324462890625;0.40619450787432087590644869123934768140316009521484375;0.71421131115999780814007635854068212211132049560546875;0.468808289855592585926302717780345119535923004150390625;0.58698714603750146157068456886918283998966217041015625]
      mask Display: e = 0.06;c1 = [120 150 230]/255;c2 = ([120 150 230]+0)/383;c3 = ([120 150 230]+128)/383;patch([0 1 1 0],[0 0 1 1],c1);patch([0 1 1 1-e 1-e 0+e],[0 0 1 1-e 0+e 0+e],c2);patch([0 0 1 1-e 0+e 0+e],[0 1 1 1-e 1-e 0+e],c3);plot([0 1 1 0 0],[0 0 1 1 0]);disp('weights');
  "IW{2,1}(97,:)'" : Constant  Value=[1.282711354094460798336285733967088162899017333984375;-0.5914293341576228879574728125589899718761444091796875;0.1711292838626052859041237752535380423069000244140625;1.46069495716096842130582444951869547367095947265625;1.604770532067913091367472588899545371532440185546875;-0.205326773636084591867501103479298762977123260498046875;0.91790018131375472609789767375332303345203399658203125;1.8102428144613649241279063062393106520175933837890625]
      mask Display: e = 0.06;c1 = [120 150 230]/255;c2 = ([120 150 230]+0)/383;c3 = ([120 150 230]+128)/383;patch([0 1 1 0],[0 0 1 1],c1);patch([0 1 1 1-e 1-e 0+e],[0 0 1 1-e 0+e 0+e],c2);patch([0 0 1 1-e 0+e 0+e],[0 1 1 1-e 1-e 0+e],c3);plot([0 1 1 0 0],[0 0 1 1 0]);disp('weights');
  "IW{2,1}(970,:)'" : Constant  Value=[1.30097587495642752486446624970994889736175537109375;-1.413257400376857209067793519352562725543975830078125;1.784785979792246735087246634066104888916015625;1.3141106643294417910539095828426070511341094970703125;0.49893547576224894779528540311730466783046722412109375;-1.0279658736542176544759286116459406912326812744140625;-0.92258064701167519228164337619091384112834930419921875;0.51803054389287128689289829708286561071872711181640625]
      mask Display: e = 0.06;c1 = [120 150 230]/255;c2 = ([120 150 230]+0)/383;c3 = ([120 150 230]+128)/383;patch([0 1 1 0],[0 0 1 1],c1);patch([0 1 1 1-e 1-e 0+e],[0 0 1 1-e 0+e 0+e],c2);patch([0 0 1 1-e 0+e 0+e],[0 1 1 1-e 1-e 0+e],c3);plot([0 1 1 0 0],[0 0 1 1 0]);disp('weights');
  "IW{2,1}(971,:)'" : Constant  Value=[1.70008261798046245161231126985512673854827880859375;0.346576994365216328741752249698038212954998016357421875;1.351918623248673068104608319117687642574310302734375;1.345828453666604307414900176809169352054595947265625;-0.19050224560682604835193387771141715347766876220703125;-1.0027599549271812851003460309584625065326690673828125;-1.813858803072877723394640270271338522434234619140625;-0.1789809936350310604069591136067174375057220458984375]
      mask Display: e = 0.06;c1 = [120 150 230]/255;c2 = ([120 150 230]+0)/383;c3 = ([120 150 230]+128)/383;patch([0 1 1 0],[0 0 1 1],c1);patch([0 1 1 1-e 1-e 0+e],[0 0 1 1-e 0+e 0+e],c2);patch([0 0 1 1-e 0+e 0+e],[0 1 1 1-e 1-e 0+e],c3);plot([0 1 1 0 0],[0 0 1 1 0]);disp('weights');
  "IW{2,1}(972,:)'" : Constant  Value=[1.596318832479507676680441363714635372161865234375;1.0267673420422005481356109157786704599857330322265625;0.0080212241673329465196928822479094378650188446044921875;-1.0752614192178866492355382433743216097354888916015625;-0.5243409963553820052339915491756983101367950439453125;-0.8748589559395159032106903396197594702243804931640625;1.1828231043354069385031834826804697513580322265625;-1.9440588251773143202427718279068358242511749267578125]
      mask Display: e = 0.06;c1 = [120 150 230]/255;c2 = ([120 150 230]+0)/383;c3 = ([120 150 230]+128)/383;patch([0 1 1 0],[0 0 1 1],c1);patch([0 1 1 1-e 1-e 0+e],[0 0 1 1-e 0+e 0+e],c2);patch([0 0 1 1-e 0+e 0+e],[0 1 1 1-e 1-e 0+e],c3);plot([0 1 1 0 0],[0 0 1 1 0]);disp('weights');
  "IW{2,1}(973,:)'" : Constant  Value=[-0.88587318254677105411332149742520414292812347412109375;0.448863905225653780917127733118832111358642578125;1.967483958518759568079303790000267326831817626953125;0.36780351762035923268712167555349878966808319091796875;0.8947873257794720647240183097892440855503082275390625;0.77218989045748409605351980644627474248409271240234375;0.7454918077668575282501706169568933546543121337890625;2.0464112355018766464809232275001704692840576171875]
      mask Display: e = 0.06;c1 = [120 150 230]/255;c2 = ([120 150 230]+0)/383;c3 = ([120 150 230]+128)/383;patch([0 1 1 0],[0 0 1 1],c1);patch([0 1 1 1-e 1-e 0+e],[0 0 1 1-e 0+e 0+e],c2);patch([0 0 1 1-e 0+e 0+e],[0 1 1 1-e 1-e 0+e],c3);plot([0 1 1 0 0],[0 0 1 1 0]);disp('weights');
  "IW{2,1}(974,:)'" : Constant  Value=[0.99745527051682059127557522515417076647281646728515625;1.7164361321599788112735041067935526371002197265625;0.0940270418476275293695465506971231661736965179443359375;-0.10765806024845316068994094393929117359220981597900390625;-1.2933797556933084305086367749026976525783538818359375;1.434425122428995447165789300925098359584808349609375;-1.8168069226142498084897169974283315241336822509765625;-0.24648770438352285427896504188538528978824615478515625]
      mask Display: e = 0.06;c1 = [120 150 230]/255;c2 = ([120 150 230]+0)/383;c3 = ([120 150 230]+128)/383;patch([0 1 1 0],[0 0 1 1],c1);patch([0 1 1 1-e 1-e 0+e],[0 0 1 1-e 0+e 0+e],c2);patch([0 0 1 1-e 0+e 0+e],[0 1 1 1-e 1-e 0+e],c3);plot([0 1 1 0 0],[0 0 1 1 0]);disp('weights');
  "IW{2,1}(975,:)'" : Constant  Value=[1.6943498603728344154006890676100738346576690673828125;-0.21285259154969449202354780936730094254016876220703125;-0.2814179374322007820552471457631327211856842041015625;1.9536517416272178859770747294533066451549530029296875;-0.5633710074509419296617807049187831580638885498046875;1.13667181148146756441974503104574978351593017578125;0.2383594795615215089501504053259850479662418365478515625;-1.5959243038666157676885859473259188234806060791015625]
      mask Display: e = 0.06;c1 = [120 150 230]/255;c2 = ([120 150 230]+0)/383;c3 = ([120 150 230]+128)/383;patch([0 1 1 0],[0 0 1 1],c1);patch([0 1 1 1-e 1-e 0+e],[0 0 1 1-e 0+e 0+e],c2);patch([0 0 1 1-e 0+e 0+e],[0 1 1 1-e 1-e 0+e],c3);plot([0 1 1 0 0],[0 0 1 1 0]);disp('weights');
  "IW{2,1}(976,:)'" : Constant  Value=[-1.430442378821195514859709874144755303859710693359375;0.83201097605623675068642342012026347219944000244140625;1.2950231210869345144232056554756127297878265380859375;0.75113644041946991958269563838257454335689544677734375;-1.29809887590576966687194726546294987201690673828125;-0.88599296863452214889633751226938329637050628662109375;0.61433804719081930301172178587876260280609130859375;-1.7871750276185778272264315091888420283794403076171875]
      mask Display: e = 0.06;c1 = [120 150 230]/255;c2 = ([120 150 230]+0)/383;c3 = ([120 150 230]+128)/383;patch([0 1 1 0],[0 0 1 1],c1);patch([0 1 1 1-e 1-e 0+e],[0 0 1 1-e 0+e 0+e],c2);patch([0 0 1 1-e 0+e 0+e],[0 1 1 1-e 1-e 0+e],c3);plot([0 1 1 0 0],[0 0 1 1 0]);disp('weights');
  "IW{2,1}(977,:)'" : Constant  Value=[-0.1945978955927430698036317835430963896214962005615234375;-0.61269401246829968687990231046569533646106719970703125;1.8306762470354656091586775801260955631732940673828125;0.76605343241544687771238386631011962890625;1.0920580171095781718548778371769003570079803466796875;-1.221035346876404137361760149360634386539459228515625;-1.3234282501912904006502458287286572158336639404296875;-1.4891973903592738981416232491028495132923126220703125]
      mask Display: e = 0.06;c1 = [120 150 230]/255;c2 = ([120 150 230]+0)/383;c3 = ([120 150 230]+128)/383;patch([0 1 1 0],[0 0 1 1],c1);patch([0 1 1 1-e 1-e 0+e],[0 0 1 1-e 0+e 0+e],c2);patch([0 0 1 1-e 0+e 0+e],[0 1 1 1-e 1-e 0+e],c3);plot([0 1 1 0 0],[0 0 1 1 0]);disp('weights');
  "IW{2,1}(978,:)'" : Constant  Value=[0.51735263737015502183425041948794387280941009521484375;-0.5265140858587933347934040284599177539348602294921875;0.7357169311985345405702219068189151585102081298828125;2.7581288521162701243838455411605536937713623046875;0.2249976228693003343916956282555474899709224700927734375;-0.270958692618770979887443672851077280938625335693359375;0.33713704342140837777463957536383531987667083740234375;-1.4460329662342534806640514943865127861499786376953125]
      mask Display: e = 0.06;c1 = [120 150 230]/255;c2 = ([120 150 230]+0)/383;c3 = ([120 150 230]+128)/383;patch([0 1 1 0],[0 0 1 1],c1);patch([0 1 1 1-e 1-e 0+e],[0 0 1 1-e 0+e 0+e],c2);patch([0 0 1 1-e 0+e 0+e],[0 1 1 1-e 1-e 0+e],c3);plot([0 1 1 0 0],[0 0 1 1 0]);disp('weights');
  "IW{2,1}(979,:)'" : Constant  Value=[-0.4973972287288412896799627560540102422237396240234375;1.2815740057532269968731952758389525115489959716796875;-1.2453805802750768094711020239628851413726806640625;-0.75807584719449050414397106578689999878406524658203125;2.11309911531509708737530672806315124034881591796875;-1.3830651254209624934077282887301407754421234130859375;0.2942661431060746846100073526031337678432464599609375;0.79506676739427939448745519257499836385250091552734375]
      mask Display: e = 0.06;c1 = [120 150 230]/255;c2 = ([120 150 230]+0)/383;c3 = ([120 150 230]+128)/383;patch([0 1 1 0],[0 0 1 1],c1);patch([0 1 1 1-e 1-e 0+e],[0 0 1 1-e 0+e 0+e],c2);patch([0 0 1 1-e 0+e 0+e],[0 1 1 1-e 1-e 0+e],c3);plot([0 1 1 0 0],[0 0 1 1 0]);disp('weights');
  "IW{2,1}(98,:)'" : Constant  Value=[1.48793763146858282198081724345684051513671875;-0.274553674905285094443030402544536627829074859619140625;-0.77815930263741572847635552534484304487705230712890625;-0.67707310116150531964507308657630346715450286865234375;-1.2095201972653406574664813888375647366046905517578125;-2.0081002653242450151083176024258136749267578125;0.95627496907814457660634843705338425934314727783203125;-1.119875173839086190952230026596225798130035400390625]
      mask Display: e = 0.06;c1 = [120 150 230]/255;c2 = ([120 150 230]+0)/383;c3 = ([120 150 230]+128)/383;patch([0 1 1 0],[0 0 1 1],c1);patch([0 1 1 1-e 1-e 0+e],[0 0 1 1-e 0+e 0+e],c2);patch([0 0 1 1-e 0+e 0+e],[0 1 1 1-e 1-e 0+e],c3);plot([0 1 1 0 0],[0 0 1 1 0]);disp('weights');
  "IW{2,1}(980,:)'" : Constant  Value=[-0.777505871882129273586770068504847586154937744140625;-1.813749485632772273646651228773407638072967529296875;0.65458867504490936273242596143973059952259063720703125;-0.97945478349737025158816550174378789961338043212890625;-1.35898229702817818775884006754495203495025634765625;-1.9080369881059493497588164245826192200183868408203125;0.1447312105305710028257948351892991922795772552490234375;-0.48212346322430066347664023851393721997737884521484375]
      mask Display: e = 0.06;c1 = [120 150 230]/255;c2 = ([120 150 230]+0)/383;c3 = ([120 150 230]+128)/383;patch([0 1 1 0],[0 0 1 1],c1);patch([0 1 1 1-e 1-e 0+e],[0 0 1 1-e 0+e 0+e],c2);patch([0 0 1 1-e 0+e 0+e],[0 1 1 1-e 1-e 0+e],c3);plot([0 1 1 0 0],[0 0 1 1 0]);disp('weights');
  "IW{2,1}(981,:)'" : Constant  Value=[-1.5171946748330906729052003356628119945526123046875;1.026369566660863430485051139839924871921539306640625;-1.4019882602532611759471592449699528515338897705078125;0.75184421643296028836545019657933153212070465087890625;1.0309147281701640519457896516541950404644012451171875;0.955081072062122782284632194205187261104583740234375;0.3696958406381429806941696369904093444347381591796875;1.6884312546675943611518277975847013294696807861328125]
      mask Display: e = 0.06;c1 = [120 150 230]/255;c2 = ([120 150 230]+0)/383;c3 = ([120 150 230]+128)/383;patch([0 1 1 0],[0 0 1 1],c1);patch([0 1 1 1-e 1-e 0+e],[0 0 1 1-e 0+e 0+e],c2);patch([0 0 1 1-e 0+e 0+e],[0 1 1 1-e 1-e 0+e],c3);plot([0 1 1 0 0],[0 0 1 1 0]);disp('weights');
  "IW{2,1}(982,:)'" : Constant  Value=[1.3933432017993163665181555188610218465328216552734375;1.185455551029723775258162277168594300746917724609375;1.484573676831697497391360229812562465667724609375;-1.2713603262120301007342959564994089305400848388671875;-0.93765245345854431047172283797408454120159149169921875;-1.4007198667768989697179904396762140095233917236328125;-0.8388067360263715688262209368986077606678009033203125;0.53565086549773865964851893295417539775371551513671875]
      mask Display: e = 0.06;c1 = [120 150 230]/255;c2 = ([120 150 230]+0)/383;c3 = ([120 150 230]+128)/383;patch([0 1 1 0],[0 0 1 1],c1);patch([0 1 1 1-e 1-e 0+e],[0 0 1 1-e 0+e 0+e],c2);patch([0 0 1 1-e 0+e 0+e],[0 1 1 1-e 1-e 0+e],c3);plot([0 1 1 0 0],[0 0 1 1 0]);disp('weights');
  "IW{2,1}(983,:)'" : Constant  Value=[0.296646530555455978372947356547228991985321044921875;1.099509274014215609582834076718427240848541259765625;-0.82880359483012921995026545118889771401882171630859375;0.100078264140304351581534092474612407386302947998046875;-1.53807240897091812570351976319216191768646240234375;1.0892418025826471339456702480674721300601959228515625;1.6687998617025552317016945380601100623607635498046875;1.6420654133366949789518685065559111535549163818359375]
      mask Display: e = 0.06;c1 = [120 150 230]/255;c2 = ([120 150 230]+0)/383;c3 = ([120 150 230]+128)/383;patch([0 1 1 0],[0 0 1 1],c1);patch([0 1 1 1-e 1-e 0+e],[0 0 1 1-e 0+e 0+e],c2);patch([0 0 1 1-e 0+e 0+e],[0 1 1 1-e 1-e 0+e],c3);plot([0 1 1 0 0],[0 0 1 1 0]);disp('weights');
  "IW{2,1}(984,:)'" : Constant  Value=[-1.5870767135084147270163157372735440731048583984375;-0.759016624915431759035300274263136088848114013671875;0.84554069323980252104178134686662815511226654052734375;-1.587363155135319114918956984183751046657562255859375;-1.4446307716514181773703739963821135461330413818359375;1.5275392484592538178134191184653900563716888427734375;0.0290434605467117419597133931574717280454933643341064453125;0.51472169595338435055253967220778577029705047607421875]
      mask Display: e = 0.06;c1 = [120 150 230]/255;c2 = ([120 150 230]+0)/383;c3 = ([120 150 230]+128)/383;patch([0 1 1 0],[0 0 1 1],c1);patch([0 1 1 1-e 1-e 0+e],[0 0 1 1-e 0+e 0+e],c2);patch([0 0 1 1-e 0+e 0+e],[0 1 1 1-e 1-e 0+e],c3);plot([0 1 1 0 0],[0 0 1 1 0]);disp('weights');
  "IW{2,1}(985,:)'" : Constant  Value=[-0.91321839574910101955396157791255973279476165771484375;1.5366984923304378707342721099848859012126922607421875;1.4955715534083722229041768514434807002544403076171875;-1.3025203170273000896628445843816734850406646728515625;-1.1396567334561036322071458926075138151645660400390625;-0.60320379600902229721981484544812701642513275146484375;0.351563086407643277109258406198932789266109466552734375;1.4716841951810339939044069978990592062473297119140625]
      mask Display: e = 0.06;c1 = [120 150 230]/255;c2 = ([120 150 230]+0)/383;c3 = ([120 150 230]+128)/383;patch([0 1 1 0],[0 0 1 1],c1);patch([0 1 1 1-e 1-e 0+e],[0 0 1 1-e 0+e 0+e],c2);patch([0 0 1 1-e 0+e 0+e],[0 1 1 1-e 1-e 0+e],c3);plot([0 1 1 0 0],[0 0 1 1 0]);disp('weights');
  "IW{2,1}(986,:)'" : Constant  Value=[-0.8238903920815514592135286875418387353420257568359375;0.88767008410926229178272706121788360178470611572265625;0.405974174321034553258868982084095478057861328125;-1.3222097247806043895934635656885802745819091796875;2.225575612777243694750950453453697264194488525390625;1.32487582620051913551151301362551748752593994140625;1.1249932364668573381294436330790631473064422607421875;-0.258204471206715968634171076701022684574127197265625]
      mask Display: e = 0.06;c1 = [120 150 230]/255;c2 = ([120 150 230]+0)/383;c3 = ([120 150 230]+128)/383;patch([0 1 1 0],[0 0 1 1],c1);patch([0 1 1 1-e 1-e 0+e],[0 0 1 1-e 0+e 0+e],c2);patch([0 0 1 1-e 0+e 0+e],[0 1 1 1-e 1-e 0+e],c3);plot([0 1 1 0 0],[0 0 1 1 0]);disp('weights');
  "IW{2,1}(987,:)'" : Constant  Value=[0.54292332766931628018625133336172439157962799072265625;0.56450543195891011993836627880227752029895782470703125;-1.204381764119557107761693259817548096179962158203125;1.710437710191634597123311323230154812335968017578125;0.72612718833813250096653746368247084319591522216796875;1.5935356619066880501378591361572034657001495361328125;-0.7443553109648515242469102304312400519847869873046875;1.5521505290097106222191314373048953711986541748046875]
      mask Display: e = 0.06;c1 = [120 150 230]/255;c2 = ([120 150 230]+0)/383;c3 = ([120 150 230]+128)/383;patch([0 1 1 0],[0 0 1 1],c1);patch([0 1 1 1-e 1-e 0+e],[0 0 1 1-e 0+e 0+e],c2);patch([0 0 1 1-e 0+e 0+e],[0 1 1 1-e 1-e 0+e],c3);plot([0 1 1 0 0],[0 0 1 1 0]);disp('weights');
  "IW{2,1}(988,:)'" : Constant  Value=[0.0107119178060201512836524528893278329633176326751708984375;1.652622848914251374452533127623610198497772216796875;-0.01117574144352963781690046829453422105871140956878662109375;0.7530319521652140135614672544761560857295989990234375;1.7436259720050666377488823854946531355381011962890625;-0.389133132260264191781828913008212111890316009521484375;-0.352239968336103437263062687634374015033245086669921875;2.0994170861482341905457360553555190563201904296875]
      mask Display: e = 0.06;c1 = [120 150 230]/255;c2 = ([120 150 230]+0)/383;c3 = ([120 150 230]+128)/383;patch([0 1 1 0],[0 0 1 1],c1);patch([0 1 1 1-e 1-e 0+e],[0 0 1 1-e 0+e 0+e],c2);patch([0 0 1 1-e 0+e 0+e],[0 1 1 1-e 1-e 0+e],c3);plot([0 1 1 0 0],[0 0 1 1 0]);disp('weights');
  "IW{2,1}(989,:)'" : Constant  Value=[-1.4498089918905783246572127609397284686565399169921875;-1.99725884308253398558008484542369842529296875;-0.1367022934264936762094322375560295768082141876220703125;-0.493577100128493595487810807753703556954860687255859375;-1.9831495408999415541728694734047167003154754638671875;0.37853377901468931998607558853109367191791534423828125;0.205762128274529165761208560070372186601161956787109375;0.7442453407310301027877130763954482972621917724609375]
      mask Display: e = 0.06;c1 = [120 150 230]/255;c2 = ([120 150 230]+0)/383;c3 = ([120 150 230]+128)/383;patch([0 1 1 0],[0 0 1 1],c1);patch([0 1 1 1-e 1-e 0+e],[0 0 1 1-e 0+e 0+e],c2);patch([0 0 1 1-e 0+e 0+e],[0 1 1 1-e 1-e 0+e],c3);plot([0 1 1 0 0],[0 0 1 1 0]);disp('weights');
  "IW{2,1}(99,:)'" : Constant  Value=[1.5271080749283958422068963045603595674037933349609375;1.8718624856848029569533764515654183924198150634765625;-0.32370129951419623903774436257663182914257049560546875;-0.61602134629922866704276884775026701390743255615234375;1.707190771179954769110054257907904684543609619140625;1.0926742932132516017418311093933880329132080078125;0.6914590666269895269380185709451325237751007080078125;0.465593582516480586352969339714036323130130767822265625]
      mask Display: e = 0.06;c1 = [120 150 230]/255;c2 = ([120 150 230]+0)/383;c3 = ([120 150 230]+128)/383;patch([0 1 1 0],[0 0 1 1],c1);patch([0 1 1 1-e 1-e 0+e],[0 0 1 1-e 0+e 0+e],c2);patch([0 0 1 1-e 0+e 0+e],[0 1 1 1-e 1-e 0+e],c3);plot([0 1 1 0 0],[0 0 1 1 0]);disp('weights');
  "IW{2,1}(990,:)'" : Constant  Value=[-0.8996798934978171846665873090387322008609771728515625;-1.59626103232260252440255499095655977725982666015625;1.4328425300141904852324614694225601851940155029296875;-0.309483221329104996044634390273131430149078369140625;1.315477456512716525338646533782593905925750732421875;-0.35951490243182082640061025813338346779346466064453125;1.1145285421297419503616765723563730716705322265625;-1.573263436619675825767217247630469501018524169921875]
      mask Display: e = 0.06;c1 = [120 150 230]/255;c2 = ([120 150 230]+0)/383;c3 = ([120 150 230]+128)/383;patch([0 1 1 0],[0 0 1 1],c1);patch([0 1 1 1-e 1-e 0+e],[0 0 1 1-e 0+e 0+e],c2);patch([0 0 1 1-e 0+e 0+e],[0 1 1 1-e 1-e 0+e],c3);plot([0 1 1 0 0],[0 0 1 1 0]);disp('weights');
  "IW{2,1}(991,:)'" : Constant  Value=[0.0529200180353394944443579106518882326781749725341796875;1.6780336963560582574928048416040837764739990234375;1.6757979512291754087272011020104400813579559326171875;-1.01689873082483472899184562265872955322265625;-0.1966059222724370891821621398776187561452388763427734375;-0.48325687537477957089748770158621482551097869873046875;-2.02594628163469092640980306896381080150604248046875;0.11463311562071198945744754382758401334285736083984375]
      mask Display: e = 0.06;c1 = [120 150 230]/255;c2 = ([120 150 230]+0)/383;c3 = ([120 150 230]+128)/383;patch([0 1 1 0],[0 0 1 1],c1);patch([0 1 1 1-e 1-e 0+e],[0 0 1 1-e 0+e 0+e],c2);patch([0 0 1 1-e 0+e 0+e],[0 1 1 1-e 1-e 0+e],c3);plot([0 1 1 0 0],[0 0 1 1 0]);disp('weights');
  "IW{2,1}(992,:)'" : Constant  Value=[-2.124987943246554156218053321936167776584625244140625;-0.81613929862711220852844462569919414818286895751953125;0.39741509865890878305805244963266886770725250244140625;-0.5616377352376826781465979365748353302478790283203125;0.6064184556151623883835100059513933956623077392578125;-2.04889455110707618956666919984854757785797119140625;-0.030662073726915255178493424637053976766765117645263671875;-0.90156004512191245670038597381790168583393096923828125]
      mask Display: e = 0.06;c1 = [120 150 230]/255;c2 = ([120 150 230]+0)/383;c3 = ([120 150 230]+128)/383;patch([0 1 1 0],[0 0 1 1],c1);patch([0 1 1 1-e 1-e 0+e],[0 0 1 1-e 0+e 0+e],c2);patch([0 0 1 1-e 0+e 0+e],[0 1 1 1-e 1-e 0+e],c3);plot([0 1 1 0 0],[0 0 1 1 0]);disp('weights');
  "IW{2,1}(993,:)'" : Constant  Value=[1.8274147264766991138884577594581060111522674560546875;1.2664481086719978630839023026055656373500823974609375;1.570334164876414195788356664706952869892120361328125;-0.0234956655035992965918634212130200467072427272796630859375;1.1278483195361210800200524317915551364421844482421875;-0.734222943104609004905114488792605698108673095703125;-1.2903055361270434620024616378941573202610015869140625;-0.36568700325064062983670964968041516840457916259765625]
      mask Display: e = 0.06;c1 = [120 150 230]/255;c2 = ([120 150 230]+0)/383;c3 = ([120 150 230]+128)/383;patch([0 1 1 0],[0 0 1 1],c1);patch([0 1 1 1-e 1-e 0+e],[0 0 1 1-e 0+e 0+e],c2);patch([0 0 1 1-e 0+e 0+e],[0 1 1 1-e 1-e 0+e],c3);plot([0 1 1 0 0],[0 0 1 1 0]);disp('weights');
  "IW{2,1}(994,:)'" : Constant  Value=[-0.524027119389473217125896553625352680683135986328125;1.200842653376637425566286765388213098049163818359375;1.8155922236622459298160947582800872623920440673828125;-0.0052591311851987627978832762210004148073494434356689453125;-0.85342008214321862791251760427257977426052093505859375;1.533708842827310459000500486581586301326751708984375;-1.350828902281971277687944166245870292186737060546875;1.0356612273422598491379176266491413116455078125]
      mask Display: e = 0.06;c1 = [120 150 230]/255;c2 = ([120 150 230]+0)/383;c3 = ([120 150 230]+128)/383;patch([0 1 1 0],[0 0 1 1],c1);patch([0 1 1 1-e 1-e 0+e],[0 0 1 1-e 0+e 0+e],c2);patch([0 0 1 1-e 0+e 0+e],[0 1 1 1-e 1-e 0+e],c3);plot([0 1 1 0 0],[0 0 1 1 0]);disp('weights');
  "IW{2,1}(995,:)'" : Constant  Value=[-1.399645750238363017814435806940309703350067138671875;1.229344105669003983649645306286402046680450439453125;-1.2710192861487932258768296378548257052898406982421875;0.364585578584315450623165588694973848760128021240234375;-0.2534975371437708790978149409056641161441802978515625;1.679317825090111515606849934556521475315093994140625;1.5196297986623401587991111227893270552158355712890625;-0.83691356809328276700199467086349613964557647705078125]
      mask Display: e = 0.06;c1 = [120 150 230]/255;c2 = ([120 150 230]+0)/383;c3 = ([120 150 230]+128)/383;patch([0 1 1 0],[0 0 1 1],c1);patch([0 1 1 1-e 1-e 0+e],[0 0 1 1-e 0+e 0+e],c2);patch([0 0 1 1-e 0+e 0+e],[0 1 1 1-e 1-e 0+e],c3);plot([0 1 1 0 0],[0 0 1 1 0]);disp('weights');
  "IW{2,1}(996,:)'" : Constant  Value=[-0.5487349645666077524452930447296239435672760009765625;-0.415010144899522093187016480442252941429615020751953125;-1.162235784250594594624317323905415832996368408203125;0.011078994913631907970330559010108117945492267608642578125;-1.8442647043651907434735903734690509736537933349609375;0.466802323158724885576731367109459824860095977783203125;-2.176147039626128876221855534822680056095123291015625;-0.91746782487220956969764529276289977133274078369140625]
      mask Display: e = 0.06;c1 = [120 150 230]/255;c2 = ([120 150 230]+0)/383;c3 = ([120 150 230]+128)/383;patch([0 1 1 0],[0 0 1 1],c1);patch([0 1 1 1-e 1-e 0+e],[0 0 1 1-e 0+e 0+e],c2);patch([0 0 1 1-e 0+e 0+e],[0 1 1 1-e 1-e 0+e],c3);plot([0 1 1 0 0],[0 0 1 1 0]);disp('weights');
  "IW{2,1}(997,:)'" : Constant  Value=[0.87644585744421987794083861444960348308086395263671875;1.2702466816577431263368680447456426918506622314453125;1.6254593390138742936557036955491639673709869384765625;1.9907306191980798093510429680463857948780059814453125;0.6133295838029921842604608173132874071598052978515625;0.490574303271305300899740586828556843101978302001953125;-0.65049948939808655001826309671741910278797149658203125;-0.998957187277401459368775249458849430084228515625]
      mask Display: e = 0.06;c1 = [120 150 230]/255;c2 = ([120 150 230]+0)/383;c3 = ([120 150 230]+128)/383;patch([0 1 1 0],[0 0 1 1],c1);patch([0 1 1 1-e 1-e 0+e],[0 0 1 1-e 0+e 0+e],c2);patch([0 0 1 1-e 0+e 0+e],[0 1 1 1-e 1-e 0+e],c3);plot([0 1 1 0 0],[0 0 1 1 0]);disp('weights');
  "IW{2,1}(998,:)'" : Constant  Value=[1.0499232977192083371420494586345739662647247314453125;-0.91661989277039268575464348032255657017230987548828125;0.5560991744387460133935974226915277540683746337890625;1.63151834145321661395655610249377787113189697265625;1.30979655900507818699907147674821317195892333984375;1.364250111185502323252194400993175804615020751953125;-1.5228162089188745920154133273172192275524139404296875;-0.460360096792253259412319721377571113407611846923828125]
      mask Display: e = 0.06;c1 = [120 150 230]/255;c2 = ([120 150 230]+0)/383;c3 = ([120 150 230]+128)/383;patch([0 1 1 0],[0 0 1 1],c1);patch([0 1 1 1-e 1-e 0+e],[0 0 1 1-e 0+e 0+e],c2);patch([0 0 1 1-e 0+e 0+e],[0 1 1 1-e 1-e 0+e],c3);plot([0 1 1 0 0],[0 0 1 1 0]);disp('weights');
  "IW{2,1}(999,:)'" : Constant  Value=[-1.3045244189601579165582734276540577411651611328125;0.1760238793489652675550161120554548688232898712158203125;-1.669613515522500701848684911965392529964447021484375;-1.35325916183035932505163145833648741245269775390625;-0.036507460447722517304924849668168462812900543212890625;1.79872644313018792416869473527185618877410888671875;-0.84159172545010851873570345560437999665737152099609375;0.856068389680392005658404741552658379077911376953125]
      mask Display: e = 0.06;c1 = [120 150 230]/255;c2 = ([120 150 230]+0)/383;c3 = ([120 150 230]+128)/383;patch([0 1 1 0],[0 0 1 1],c1);patch([0 1 1 1-e 1-e 0+e],[0 0 1 1-e 0+e 0+e],c2);patch([0 0 1 1-e 0+e 0+e],[0 1 1 1-e 1-e 0+e],c3);plot([0 1 1 0 0],[0 0 1 1 0]);disp('weights');
  Mux : Mux  Inputs=1000
      mask Display: e = 0.06;c1 = [120 150 230]/255;c2 = ([120 150 230]+0)/383;c3 = ([120 150 230]+128)/383;patch([0 1 1 0],[0 0 1 1],c1);patch([0 1 1 1-e 1-e 0+e],[0 0 1 1-e 0+e 0+e],c2);patch([0 0 1 1-e 0+e 0+e],[0 1 1 1-e 1-e 0+e],c3);plot([0 1 1 0 0],[0 0 1 1 0]);disp('Mux');
  dotprod{1..1000} (1000 alike) : neural/Weight Functions/dotprod
      settings: SourceProductName=MATLAB Runtime - Deep Learning Toolbox  SourceProductBaseCode=Missing
  "lz{2,1}" : Outport
      mask Display: e = 0.06;c1 = [120 230 180]/255;c2 = ([120 230 180]+0)/(256+128);c3 = ([120 230 180]+128)/(256+128);patch([0 1 1 0],[0 0 1 1],c1);patch([0 1 1 1-e 1-e 0+e],[0 0 1 1-e 0+e 0+e],c2);patch([0 0 1 1-e 0+e 0+e],[0 1 1 1-e 1-e 0+e],c3);plot([0 1 1 0 0],[0 0 1 1 0]);
  wires:
  Mux/1 -> "lz{2,1}"/1
  dotprod1000/1 -> Mux/1000
  "IW{2,1}(1000,:)'"/1 -> dotprod1000/1
  dotprod999/1 -> Mux/999
  "IW{2,1}(999,:)'"/1 -> dotprod999/1
  dotprod998/1 -> Mux/998
  "IW{2,1}(998,:)'"/1 -> dotprod998/1
  dotprod997/1 -> Mux/997
  "IW{2,1}(997,:)'"/1 -> dotprod997/1
  dotprod996/1 -> Mux/996
  "IW{2,1}(996,:)'"/1 -> dotprod996/1
  dotprod995/1 -> Mux/995
  "IW{2,1}(995,:)'"/1 -> dotprod995/1
  dotprod994/1 -> Mux/994
  "IW{2,1}(994,:)'"/1 -> dotprod994/1
  dotprod993/1 -> Mux/993
  "IW{2,1}(993,:)'"/1 -> dotprod993/1
  dotprod992/1 -> Mux/992
  "IW{2,1}(992,:)'"/1 -> dotprod992/1
  dotprod991/1 -> Mux/991
  "IW{2,1}(991,:)'"/1 -> dotprod991/1
  dotprod990/1 -> Mux/990
  "IW{2,1}(990,:)'"/1 -> dotprod990/1
  dotprod989/1 -> Mux/989
  "IW{2,1}(989,:)'"/1 -> dotprod989/1
  dotprod988/1 -> Mux/988
  "IW{2,1}(988,:)'"/1 -> dotprod988/1
  dotprod987/1 -> Mux/987
  "IW{2,1}(987,:)'"/1 -> dotprod987/1
  dotprod986/1 -> Mux/986
  "IW{2,1}(986,:)'"/1 -> dotprod986/1
  dotprod985/1 -> Mux/985
  "IW{2,1}(985,:)'"/1 -> dotprod985/1
  dotprod984/1 -> Mux/984
  "IW{2,1}(984,:)'"/1 -> dotprod984/1
  dotprod983/1 -> Mux/983
  "IW{2,1}(983,:)'"/1 -> dotprod983/1
  dotprod982/1 -> Mux/982
  "IW{2,1}(982,:)'"/1 -> dotprod982/1
  dotprod981/1 -> Mux/981
  "IW{2,1}(981,:)'"/1 -> dotprod981/1
  dotprod980/1 -> Mux/980
  "IW{2,1}(980,:)'"/1 -> dotprod980/1
  dotprod979/1 -> Mux/979
  "IW{2,1}(979,:)'"/1 -> dotprod979/1
  dotprod978/1 -> Mux/978
  "IW{2,1}(978,:)'"/1 -> dotprod978/1
  dotprod977/1 -> Mux/977
  "IW{2,1}(977,:)'"/1 -> dotprod977/1
  dotprod976/1 -> Mux/976
  "IW{2,1}(976,:)'"/1 -> dotprod976/1
  dotprod975/1 -> Mux/975
  "IW{2,1}(975,:)'"/1 -> dotprod975/1
  dotprod974/1 -> Mux/974
  "IW{2,1}(974,:)'"/1 -> dotprod974/1
  dotprod973/1 -> Mux/973
  "IW{2,1}(973,:)'"/1 -> dotprod973/1
  dotprod972/1 -> Mux/972
  "IW{2,1}(972,:)'"/1 -> dotprod972/1
  dotprod971/1 -> Mux/971
  "IW{2,1}(971,:)'"/1 -> dotprod971/1
  dotprod970/1 -> Mux/970
  "IW{2,1}(970,:)'"/1 -> dotprod970/1
  dotprod969/1 -> Mux/969
  "IW{2,1}(969,:)'"/1 -> dotprod969/1
  dotprod968/1 -> Mux/968
  "IW{2,1}(968,:)'"/1 -> dotprod968/1
  dotprod967/1 -> Mux/967
  "IW{2,1}(967,:)'"/1 -> dotprod967/1
  dotprod966/1 -> Mux/966
  "IW{2,1}(966,:)'"/1 -> dotprod966/1
  dotprod965/1 -> Mux/965
  "IW{2,1}(965,:)'"/1 -> dotprod965/1
  dotprod964/1 -> Mux/964
  "IW{2,1}(964,:)'"/1 -> dotprod964/1
  dotprod963/1 -> Mux/963
  "IW{2,1}(963,:)'"/1 -> dotprod963/1
  dotprod962/1 -> Mux/962
  "IW{2,1}(962,:)'"/1 -> dotprod962/1
  dotprod961/1 -> Mux/961
  "IW{2,1}(961,:)'"/1 -> dotprod961/1
  dotprod960/1 -> Mux/960
  "IW{2,1}(960,:)'"/1 -> dotprod960/1
  dotprod959/1 -> Mux/959
  "IW{2,1}(959,:)'"/1 -> dotprod959/1
  dotprod958/1 -> Mux/958
  "IW{2,1}(958,:)'"/1 -> dotprod958/1
  dotprod957/1 -> Mux/957
  "IW{2,1}(957,:)'"/1 -> dotprod957/1
  dotprod956/1 -> Mux/956
  "IW{2,1}(956,:)'"/1 -> dotprod956/1
  dotprod955/1 -> Mux/955
  "IW{2,1}(955,:)'"/1 -> dotprod955/1
  dotprod954/1 -> Mux/954
  "IW{2,1}(954,:)'"/1 -> dotprod954/1
  dotprod953/1 -> Mux/953
  "IW{2,1}(953,:)'"/1 -> dotprod953/1
  dotprod952/1 -> Mux/952
  "IW{2,1}(952,:)'"/1 -> dotprod952/1
  dotprod951/1 -> Mux/951
  "IW{2,1}(951,:)'"/1 -> dotprod951/1
  dotprod950/1 -> Mux/950
  "IW{2,1}(950,:)'"/1 -> dotprod950/1
  dotprod949/1 -> Mux/949
  "IW{2,1}(949,:)'"/1 -> dotprod949/1
  dotprod948/1 -> Mux/948
  "IW{2,1}(948,:)'"/1 -> dotprod948/1
  dotprod947/1 -> Mux/947
  "IW{2,1}(947,:)'"/1 -> dotprod947/1
  dotprod946/1 -> Mux/946
  "IW{2,1}(946,:)'"/1 -> dotprod946/1
  dotprod945/1 -> Mux/945
  "IW{2,1}(945,:)'"/1 -> dotprod945/1
  dotprod944/1 -> Mux/944
  "IW{2,1}(944,:)'"/1 -> dotprod944/1
  dotprod943/1 -> Mux/943
  "IW{2,1}(943,:)'"/1 -> dotprod943/1
  dotprod942/1 -> Mux/942
  "IW{2,1}(942,:)'"/1 -> dotprod942/1
  dotprod941/1 -> Mux/941
  "IW{2,1}(941,:)'"/1 -> dotprod941/1
  dotprod940/1 -> Mux/940
  "IW{2,1}(940,:)'"/1 -> dotprod940/1
  dotprod939/1 -> Mux/939
  "IW{2,1}(939,:)'"/1 -> dotprod939/1
  dotprod938/1 -> Mux/938
  "IW{2,1}(938,:)'"/1 -> dotprod938/1
  dotprod937/1 -> Mux/937
  "IW{2,1}(937,:)'"/1 -> dotprod937/1
  dotprod936/1 -> Mux/936
  "IW{2,1}(936,:)'"/1 -> dotprod936/1
  dotprod935/1 -> Mux/935
  "IW{2,1}(935,:)'"/1 -> dotprod935/1
  dotprod934/1 -> Mux/934
  "IW{2,1}(934,:)'"/1 -> dotprod934/1
  dotprod933/1 -> Mux/933
  "IW{2,1}(933,:)'"/1 -> dotprod933/1
  dotprod932/1 -> Mux/932
  "IW{2,1}(932,:)'"/1 -> dotprod932/1
  dotprod931/1 -> Mux/931
  "IW{2,1}(931,:)'"/1 -> dotprod931/1
  dotprod930/1 -> Mux/930
  "IW{2,1}(930,:)'"/1 -> dotprod930/1
  dotprod929/1 -> Mux/929
  "IW{2,1}(929,:)'"/1 -> dotprod929/1
  dotprod928/1 -> Mux/928
  "IW{2,1}(928,:)'"/1 -> dotprod928/1
  dotprod927/1 -> Mux/927
  "IW{2,1}(927,:)'"/1 -> dotprod927/1
  dotprod926/1 -> Mux/926
  "IW{2,1}(926,:)'"/1 -> dotprod926/1
  dotprod925/1 -> Mux/925
  "IW{2,1}(925,:)'"/1 -> dotprod925/1
  dotprod924/1 -> Mux/924
  "IW{2,1}(924,:)'"/1 -> dotprod924/1
  dotprod923/1 -> Mux/923
  "IW{2,1}(923,:)'"/1 -> dotprod923/1
  dotprod922/1 -> Mux/922
  "IW{2,1}(922,:)'"/1 -> dotprod922/1
  dotprod921/1 -> Mux/921
  "IW{2,1}(921,:)'"/1 -> dotprod921/1
  dotprod920/1 -> Mux/920
  "IW{2,1}(920,:)'"/1 -> dotprod920/1
  dotprod919/1 -> Mux/919
  "IW{2,1}(919,:)'"/1 -> dotprod919/1
  dotprod918/1 -> Mux/918
  "IW{2,1}(918,:)'"/1 -> dotprod918/1
  dotprod917/1 -> Mux/917
  "IW{2,1}(917,:)'"/1 -> dotprod917/1
  dotprod916/1 -> Mux/916
  "IW{2,1}(916,:)'"/1 -> dotprod916/1
  dotprod915/1 -> Mux/915
  "IW{2,1}(915,:)'"/1 -> dotprod915/1
  dotprod914/1 -> Mux/914
  "IW{2,1}(914,:)'"/1 -> dotprod914/1
  dotprod913/1 -> Mux/913
  "IW{2,1}(913,:)'"/1 -> dotprod913/1
  dotprod912/1 -> Mux/912
  "IW{2,1}(912,:)'"/1 -> dotprod912/1
  dotprod911/1 -> Mux/911
  "IW{2,1}(911,:)'"/1 -> dotprod911/1
  dotprod910/1 -> Mux/910
  "IW{2,1}(910,:)'"/1 -> dotprod910/1
  dotprod909/1 -> Mux/909
  "IW{2,1}(909,:)'"/1 -> dotprod909/1
  dotprod908/1 -> Mux/908
  "IW{2,1}(908,:)'"/1 -> dotprod908/1
  dotprod907/1 -> Mux/907
  "IW{2,1}(907,:)'"/1 -> dotprod907/1
  dotprod906/1 -> Mux/906
  "IW{2,1}(906,:)'"/1 -> dotprod906/1
  dotprod905/1 -> Mux/905
  "IW{2,1}(905,:)'"/1 -> dotprod905/1
  dotprod904/1 -> Mux/904
  "IW{2,1}(904,:)'"/1 -> dotprod904/1
  dotprod903/1 -> Mux/903
  "IW{2,1}(903,:)'"/1 -> dotprod903/1
  dotprod902/1 -> Mux/902
  "IW{2,1}(902,:)'"/1 -> dotprod902/1
  dotprod901/1 -> Mux/901
  "IW{2,1}(901,:)'"/1 -> dotprod901/1
  dotprod900/1 -> Mux/900
  "IW{2,1}(900,:)'"/1 -> dotprod900/1
  dotprod899/1 -> Mux/899
  "IW{2,1}(899,:)'"/1 -> dotprod899/1
  dotprod898/1 -> Mux/898
  "IW{2,1}(898,:)'"/1 -> dotprod898/1
  dotprod897/1 -> Mux/897
  "IW{2,1}(897,:)'"/1 -> dotprod897/1
  dotprod896/1 -> Mux/896
  "IW{2,1}(896,:)'"/1 -> dotprod896/1
  dotprod895/1 -> Mux/895
  "IW{2,1}(895,:)'"/1 -> dotprod895/1
  dotprod894/1 -> Mux/894
  "IW{2,1}(894,:)'"/1 -> dotprod894/1
  dotprod893/1 -> Mux/893
  "IW{2,1}(893,:)'"/1 -> dotprod893/1
  dotprod892/1 -> Mux/892
  "IW{2,1}(892,:)'"/1 -> dotprod892/1
  dotprod891/1 -> Mux/891
  "IW{2,1}(891,:)'"/1 -> dotprod891/1
  dotprod890/1 -> Mux/890
  "IW{2,1}(890,:)'"/1 -> dotprod890/1
  dotprod889/1 -> Mux/889
  "IW{2,1}(889,:)'"/1 -> dotprod889/1
  dotprod888/1 -> Mux/888
  "IW{2,1}(888,:)'"/1 -> dotprod888/1
  dotprod887/1 -> Mux/887
  "IW{2,1}(887,:)'"/1 -> dotprod887/1
  dotprod886/1 -> Mux/886
  "IW{2,1}(886,:)'"/1 -> dotprod886/1
  dotprod885/1 -> Mux/885
  "IW{2,1}(885,:)'"/1 -> dotprod885/1
  dotprod884/1 -> Mux/884
  "IW{2,1}(884,:)'"/1 -> dotprod884/1
  dotprod883/1 -> Mux/883
  "IW{2,1}(883,:)'"/1 -> dotprod883/1
  dotprod882/1 -> Mux/882
  "IW{2,1}(882,:)'"/1 -> dotprod882/1
  dotprod881/1 -> Mux/881
  "IW{2,1}(881,:)'"/1 -> dotprod881/1
  dotprod880/1 -> Mux/880
  "IW{2,1}(880,:)'"/1 -> dotprod880/1
  dotprod879/1 -> Mux/879
  "IW{2,1}(879,:)'"/1 -> dotprod879/1
  dotprod878/1 -> Mux/878
  "IW{2,1}(878,:)'"/1 -> dotprod878/1
  dotprod877/1 -> Mux/877
  "IW{2,1}(877,:)'"/1 -> dotprod877/1
  dotprod876/1 -> Mux/876
  "IW{2,1}(876,:)'"/1 -> dotprod876/1
  dotprod875/1 -> Mux/875
  "IW{2,1}(875,:)'"/1 -> dotprod875/1
  dotprod874/1 -> Mux/874
  "IW{2,1}(874,:)'"/1 -> dotprod874/1
  dotprod873/1 -> Mux/873
  "IW{2,1}(873,:)'"/1 -> dotprod873/1
  dotprod872/1 -> Mux/872
  "IW{2,1}(872,:)'"/1 -> dotprod872/1
  dotprod871/1 -> Mux/871
  "IW{2,1}(871,:)'"/1 -> dotprod871/1
  dotprod870/1 -> Mux/870
  "IW{2,1}(870,:)'"/1 -> dotprod870/1
  dotprod869/1 -> Mux/869
  "IW{2,1}(869,:)'"/1 -> dotprod869/1
  dotprod868/1 -> Mux/868
  "IW{2,1}(868,:)'"/1 -> dotprod868/1
  dotprod867/1 -> Mux/867
  "IW{2,1}(867,:)'"/1 -> dotprod867/1
  dotprod866/1 -> Mux/866
  "IW{2,1}(866,:)'"/1 -> dotprod866/1
  dotprod865/1 -> Mux/865
  "IW{2,1}(865,:)'"/1 -> dotprod865/1
  dotprod864/1 -> Mux/864
  "IW{2,1}(864,:)'"/1 -> dotprod864/1
  dotprod863/1 -> Mux/863
  "IW{2,1}(863,:)'"/1 -> dotprod863/1
  dotprod862/1 -> Mux/862
  "IW{2,1}(862,:)'"/1 -> dotprod862/1
  dotprod861/1 -> Mux/861
  "IW{2,1}(861,:)'"/1 -> dotprod861/1
  dotprod860/1 -> Mux/860
  "IW{2,1}(860,:)'"/1 -> dotprod860/1
  dotprod859/1 -> Mux/859
  "IW{2,1}(859,:)'"/1 -> dotprod859/1
  dotprod858/1 -> Mux/858
  "IW{2,1}(858,:)'"/1 -> dotprod858/1
  dotprod857/1 -> Mux/857
  "IW{2,1}(857,:)'"/1 -> dotprod857/1
  dotprod856/1 -> Mux/856
  "IW{2,1}(856,:)'"/1 -> dotprod856/1
  dotprod855/1 -> Mux/855
  "IW{2,1}(855,:)'"/1 -> dotprod855/1
  dotprod854/1 -> Mux/854
  "IW{2,1}(854,:)'"/1 -> dotprod854/1
  dotprod853/1 -> Mux/853
  "IW{2,1}(853,:)'"/1 -> dotprod853/1
  dotprod852/1 -> Mux/852
  "IW{2,1}(852,:)'"/1 -> dotprod852/1
  dotprod851/1 -> Mux/851
  "IW{2,1}(851,:)'"/1 -> dotprod851/1
  dotprod850/1 -> Mux/850
  "IW{2,1}(850,:)'"/1 -> dotprod850/1
  dotprod849/1 -> Mux/849
  "IW{2,1}(849,:)'"/1 -> dotprod849/1
  dotprod848/1 -> Mux/848
  "IW{2,1}(848,:)'"/1 -> dotprod848/1
  dotprod847/1 -> Mux/847
  "IW{2,1}(847,:)'"/1 -> dotprod847/1
  dotprod846/1 -> Mux/846
  "IW{2,1}(846,:)'"/1 -> dotprod846/1
  dotprod845/1 -> Mux/845
  "IW{2,1}(845,:)'"/1 -> dotprod845/1
  dotprod844/1 -> Mux/844
  "IW{2,1}(844,:)'"/1 -> dotprod844/1
  dotprod843/1 -> Mux/843
  "IW{2,1}(843,:)'"/1 -> dotprod843/1
  dotprod842/1 -> Mux/842
  "IW{2,1}(842,:)'"/1 -> dotprod842/1
  dotprod841/1 -> Mux/841
  "IW{2,1}(841,:)'"/1 -> dotprod841/1
  dotprod840/1 -> Mux/840
  "IW{2,1}(840,:)'"/1 -> dotprod840/1
  dotprod839/1 -> Mux/839
  "IW{2,1}(839,:)'"/1 -> dotprod839/1
  dotprod838/1 -> Mux/838
  "IW{2,1}(838,:)'"/1 -> dotprod838/1
  dotprod837/1 -> Mux/837
  "IW{2,1}(837,:)'"/1 -> dotprod837/1
  dotprod836/1 -> Mux/836
  "IW{2,1}(836,:)'"/1 -> dotprod836/1
  dotprod835/1 -> Mux/835
  "IW{2,1}(835,:)'"/1 -> dotprod835/1
  dotprod834/1 -> Mux/834
  "IW{2,1}(834,:)'"/1 -> dotprod834/1
  dotprod833/1 -> Mux/833
  "IW{2,1}(833,:)'"/1 -> dotprod833/1
  dotprod832/1 -> Mux/832
  "IW{2,1}(832,:)'"/1 -> dotprod832/1
  dotprod831/1 -> Mux/831
  "IW{2,1}(831,:)'"/1 -> dotprod831/1
  dotprod830/1 -> Mux/830
  "IW{2,1}(830,:)'"/1 -> dotprod830/1
  dotprod829/1 -> Mux/829
  "IW{2,1}(829,:)'"/1 -> dotprod829/1
  dotprod828/1 -> Mux/828
  "IW{2,1}(828,:)'"/1 -> dotprod828/1
  dotprod827/1 -> Mux/827
  "IW{2,1}(827,:)'"/1 -> dotprod827/1
  dotprod826/1 -> Mux/826
  "IW{2,1}(826,:)'"/1 -> dotprod826/1
  dotprod825/1 -> Mux/825
  "IW{2,1}(825,:)'"/1 -> dotprod825/1
  dotprod824/1 -> Mux/824
  "IW{2,1}(824,:)'"/1 -> dotprod824/1
  dotprod823/1 -> Mux/823
  "IW{2,1}(823,:)'"/1 -> dotprod823/1
  dotprod822/1 -> Mux/822
  "IW{2,1}(822,:)'"/1 -> dotprod822/1
  dotprod821/1 -> Mux/821
  "IW{2,1}(821,:)'"/1 -> dotprod821/1
  dotprod820/1 -> Mux/820
  "IW{2,1}(820,:)'"/1 -> dotprod820/1
  dotprod819/1 -> Mux/819
  "IW{2,1}(819,:)'"/1 -> dotprod819/1
  dotprod818/1 -> Mux/818
  "IW{2,1}(818,:)'"/1 -> dotprod818/1
  dotprod817/1 -> Mux/817
  "IW{2,1}(817,:)'"/1 -> dotprod817/1
  dotprod816/1 -> Mux/816
  "IW{2,1}(816,:)'"/1 -> dotprod816/1
  dotprod815/1 -> Mux/815
  "IW{2,1}(815,:)'"/1 -> dotprod815/1
  dotprod814/1 -> Mux/814
  "IW{2,1}(814,:)'"/1 -> dotprod814/1
  dotprod813/1 -> Mux/813
  "IW{2,1}(813,:)'"/1 -> dotprod813/1
  dotprod812/1 -> Mux/812
  "IW{2,1}(812,:)'"/1 -> dotprod812/1
  dotprod811/1 -> Mux/811
  "IW{2,1}(811,:)'"/1 -> dotprod811/1
  dotprod810/1 -> Mux/810
  "IW{2,1}(810,:)'"/1 -> dotprod810/1
  dotprod809/1 -> Mux/809
  "IW{2,1}(809,:)'"/1 -> dotprod809/1
  dotprod808/1 -> Mux/808
  "IW{2,1}(808,:)'"/1 -> dotprod808/1
  dotprod807/1 -> Mux/807
  "IW{2,1}(807,:)'"/1 -> dotprod807/1
  dotprod806/1 -> Mux/806
  "IW{2,1}(806,:)'"/1 -> dotprod806/1
  dotprod805/1 -> Mux/805
  "IW{2,1}(805,:)'"/1 -> dotprod805/1
  dotprod804/1 -> Mux/804
  "IW{2,1}(804,:)'"/1 -> dotprod804/1
  dotprod803/1 -> Mux/803
  "IW{2,1}(803,:)'"/1 -> dotprod803/1
  dotprod802/1 -> Mux/802
  "IW{2,1}(802,:)'"/1 -> dotprod802/1
  dotprod801/1 -> Mux/801
  "IW{2,1}(801,:)'"/1 -> dotprod801/1
  dotprod800/1 -> Mux/800
  "IW{2,1}(800,:)'"/1 -> dotprod800/1
  dotprod799/1 -> Mux/799
  "IW{2,1}(799,:)'"/1 -> dotprod799/1
  dotprod798/1 -> Mux/798
  "IW{2,1}(798,:)'"/1 -> dotprod798/1
  dotprod797/1 -> Mux/797
  "IW{2,1}(797,:)'"/1 -> dotprod797/1
  dotprod796/1 -> Mux/796
  "IW{2,1}(796,:)'"/1 -> dotprod796/1
  dotprod795/1 -> Mux/795
  "IW{2,1}(795,:)'"/1 -> dotprod795/1
  dotprod794/1 -> Mux/794
  "IW{2,1}(794,:)'"/1 -> dotprod794/1
  dotprod793/1 -> Mux/793
  "IW{2,1}(793,:)'"/1 -> dotprod793/1
  dotprod792/1 -> Mux/792
  "IW{2,1}(792,:)'"/1 -> dotprod792/1
  dotprod791/1 -> Mux/791
  "IW{2,1}(791,:)'"/1 -> dotprod791/1
  dotprod790/1 -> Mux/790
  "IW{2,1}(790,:)'"/1 -> dotprod790/1
  dotprod789/1 -> Mux/789
  "IW{2,1}(789,:)'"/1 -> dotprod789/1
  dotprod788/1 -> Mux/788
  "IW{2,1}(788,:)'"/1 -> dotprod788/1
  dotprod787/1 -> Mux/787
  "IW{2,1}(787,:)'"/1 -> dotprod787/1
  dotprod786/1 -> Mux/786
  "IW{2,1}(786,:)'"/1 -> dotprod786/1
  dotprod785/1 -> Mux/785
  "IW{2,1}(785,:)'"/1 -> dotprod785/1
  dotprod784/1 -> Mux/784
  "IW{2,1}(784,:)'"/1 -> dotprod784/1
  dotprod783/1 -> Mux/783
  "IW{2,1}(783,:)'"/1 -> dotprod783/1
  dotprod782/1 -> Mux/782
  "IW{2,1}(782,:)'"/1 -> dotprod782/1
  dotprod781/1 -> Mux/781
  "IW{2,1}(781,:)'"/1 -> dotprod781/1
  dotprod780/1 -> Mux/780
  "IW{2,1}(780,:)'"/1 -> dotprod780/1
  dotprod779/1 -> Mux/779
  "IW{2,1}(779,:)'"/1 -> dotprod779/1
  dotprod778/1 -> Mux/778
  "IW{2,1}(778,:)'"/1 -> dotprod778/1
  dotprod777/1 -> Mux/777
  "IW{2,1}(777,:)'"/1 -> dotprod777/1
  dotprod776/1 -> Mux/776
  "IW{2,1}(776,:)'"/1 -> dotprod776/1
  dotprod775/1 -> Mux/775
  "IW{2,1}(775,:)'"/1 -> dotprod775/1
  dotprod774/1 -> Mux/774
  "IW{2,1}(774,:)'"/1 -> dotprod774/1
  dotprod773/1 -> Mux/773
  "IW{2,1}(773,:)'"/1 -> dotprod773/1
  dotprod772/1 -> Mux/772
  "IW{2,1}(772,:)'"/1 -> dotprod772/1
  dotprod771/1 -> Mux/771
  "IW{2,1}(771,:)'"/1 -> dotprod771/1
  dotprod770/1 -> Mux/770
  "IW{2,1}(770,:)'"/1 -> dotprod770/1
  dotprod769/1 -> Mux/769
  "IW{2,1}(769,:)'"/1 -> dotprod769/1
  dotprod768/1 -> Mux/768
  "IW{2,1}(768,:)'"/1 -> dotprod768/1
  dotprod767/1 -> Mux/767
  "IW{2,1}(767,:)'"/1 -> dotprod767/1
  dotprod766/1 -> Mux/766
  "IW{2,1}(766,:)'"/1 -> dotprod766/1
  dotprod765/1 -> Mux/765
  "IW{2,1}(765,:)'"/1 -> dotprod765/1
  dotprod764/1 -> Mux/764
  "IW{2,1}(764,:)'"/1 -> dotprod764/1
  dotprod763/1 -> Mux/763
  "IW{2,1}(763,:)'"/1 -> dotprod763/1
  dotprod762/1 -> Mux/762
  "IW{2,1}(762,:)'"/1 -> dotprod762/1
  dotprod761/1 -> Mux/761
  "IW{2,1}(761,:)'"/1 -> dotprod761/1
  dotprod760/1 -> Mux/760
  "IW{2,1}(760,:)'"/1 -> dotprod760/1
  dotprod759/1 -> Mux/759
  "IW{2,1}(759,:)'"/1 -> dotprod759/1
  dotprod758/1 -> Mux/758
  "IW{2,1}(758,:)'"/1 -> dotprod758/1
  dotprod757/1 -> Mux/757
  "IW{2,1}(757,:)'"/1 -> dotprod757/1
  dotprod756/1 -> Mux/756
  "IW{2,1}(756,:)'"/1 -> dotprod756/1
  dotprod755/1 -> Mux/755
  "IW{2,1}(755,:)'"/1 -> dotprod755/1
  dotprod754/1 -> Mux/754
  "IW{2,1}(754,:)'"/1 -> dotprod754/1
  dotprod753/1 -> Mux/753
  "IW{2,1}(753,:)'"/1 -> dotprod753/1
  dotprod752/1 -> Mux/752
  "IW{2,1}(752,:)'"/1 -> dotprod752/1
  dotprod751/1 -> Mux/751
  "IW{2,1}(751,:)'"/1 -> dotprod751/1
  dotprod750/1 -> Mux/750
  "IW{2,1}(750,:)'"/1 -> dotprod750/1
  dotprod749/1 -> Mux/749
  "IW{2,1}(749,:)'"/1 -> dotprod749/1
  dotprod748/1 -> Mux/748
  "IW{2,1}(748,:)'"/1 -> dotprod748/1
  dotprod747/1 -> Mux/747
  "IW{2,1}(747,:)'"/1 -> dotprod747/1
  dotprod746/1 -> Mux/746
  "IW{2,1}(746,:)'"/1 -> dotprod746/1
  dotprod745/1 -> Mux/745
  "IW{2,1}(745,:)'"/1 -> dotprod745/1
  dotprod744/1 -> Mux/744
  "IW{2,1}(744,:)'"/1 -> dotprod744/1
  dotprod743/1 -> Mux/743
  "IW{2,1}(743,:)'"/1 -> dotprod743/1
  dotprod742/1 -> Mux/742
  "IW{2,1}(742,:)'"/1 -> dotprod742/1
  dotprod741/1 -> Mux/741
  "IW{2,1}(741,:)'"/1 -> dotprod741/1
  dotprod740/1 -> Mux/740
  "IW{2,1}(740,:)'"/1 -> dotprod740/1
  dotprod739/1 -> Mux/739
  "IW{2,1}(739,:)'"/1 -> dotprod739/1
  dotprod738/1 -> Mux/738
  "IW{2,1}(738,:)'"/1 -> dotprod738/1
  dotprod737/1 -> Mux/737
  "IW{2,1}(737,:)'"/1 -> dotprod737/1
  dotprod736/1 -> Mux/736
  "IW{2,1}(736,:)'"/1 -> dotprod736/1
  dotprod735/1 -> Mux/735
  "IW{2,1}(735,:)'"/1 -> dotprod735/1
  dotprod734/1 -> Mux/734
  "IW{2,1}(734,:)'"/1 -> dotprod734/1
  dotprod733/1 -> Mux/733
  "IW{2,1}(733,:)'"/1 -> dotprod733/1
  dotprod732/1 -> Mux/732
  "IW{2,1}(732,:)'"/1 -> dotprod732/1
  dotprod731/1 -> Mux/731
  "IW{2,1}(731,:)'"/1 -> dotprod731/1
  dotprod730/1 -> Mux/730
  "IW{2,1}(730,:)'"/1 -> dotprod730/1
  dotprod729/1 -> Mux/729
  "IW{2,1}(729,:)'"/1 -> dotprod729/1
  dotprod728/1 -> Mux/728
  "IW{2,1}(728,:)'"/1 -> dotprod728/1
  dotprod727/1 -> Mux/727
  "IW{2,1}(727,:)'"/1 -> dotprod727/1
  dotprod726/1 -> Mux/726
  "IW{2,1}(726,:)'"/1 -> dotprod726/1
  dotprod725/1 -> Mux/725
  "IW{2,1}(725,:)'"/1 -> dotprod725/1
  dotprod724/1 -> Mux/724
  "IW{2,1}(724,:)'"/1 -> dotprod724/1
  dotprod723/1 -> Mux/723
  "IW{2,1}(723,:)'"/1 -> dotprod723/1
  dotprod722/1 -> Mux/722
  "IW{2,1}(722,:)'"/1 -> dotprod722/1
  dotprod721/1 -> Mux/721
  "IW{2,1}(721,:)'"/1 -> dotprod721/1
  dotprod720/1 -> Mux/720
  "IW{2,1}(720,:)'"/1 -> dotprod720/1
  dotprod719/1 -> Mux/719
  "IW{2,1}(719,:)'"/1 -> dotprod719/1
  dotprod718/1 -> Mux/718
  "IW{2,1}(718,:)'"/1 -> dotprod718/1
  dotprod717/1 -> Mux/717
  "IW{2,1}(717,:)'"/1 -> dotprod717/1
  dotprod716/1 -> Mux/716
  "IW{2,1}(716,:)'"/1 -> dotprod716/1
  dotprod715/1 -> Mux/715
  "IW{2,1}(715,:)'"/1 -> dotprod715/1
  dotprod714/1 -> Mux/714
  "IW{2,1}(714,:)'"/1 -> dotprod714/1
  dotprod713/1 -> Mux/713
  "IW{2,1}(713,:)'"/1 -> dotprod713/1
  dotprod712/1 -> Mux/712
  "IW{2,1}(712,:)'"/1 -> dotprod712/1
  dotprod711/1 -> Mux/711
  "IW{2,1}(711,:)'"/1 -> dotprod711/1
  dotprod710/1 -> Mux/710
  "IW{2,1}(710,:)'"/1 -> dotprod710/1
  dotprod709/1 -> Mux/709
  "IW{2,1}(709,:)'"/1 -> dotprod709/1
  dotprod708/1 -> Mux/708
  "IW{2,1}(708,:)'"/1 -> dotprod708/1
  dotprod707/1 -> Mux/707
  "IW{2,1}(707,:)'"/1 -> dotprod707/1
  dotprod706/1 -> Mux/706
  "IW{2,1}(706,:)'"/1 -> dotprod706/1
  dotprod705/1 -> Mux/705
  "IW{2,1}(705,:)'"/1 -> dotprod705/1
  dotprod704/1 -> Mux/704
  "IW{2,1}(704,:)'"/1 -> dotprod704/1
  dotprod703/1 -> Mux/703
  "IW{2,1}(703,:)'"/1 -> dotprod703/1
  dotprod702/1 -> Mux/702
  "IW{2,1}(702,:)'"/1 -> dotprod702/1
  dotprod701/1 -> Mux/701
  "IW{2,1}(701,:)'"/1 -> dotprod701/1
  dotprod700/1 -> Mux/700
  "IW{2,1}(700,:)'"/1 -> dotprod700/1
  dotprod699/1 -> Mux/699
  "IW{2,1}(699,:)'"/1 -> dotprod699/1
  dotprod698/1 -> Mux/698
  "IW{2,1}(698,:)'"/1 -> dotprod698/1
  dotprod697/1 -> Mux/697
  "IW{2,1}(697,:)'"/1 -> dotprod697/1
  dotprod696/1 -> Mux/696
  "IW{2,1}(696,:)'"/1 -> dotprod696/1
  dotprod695/1 -> Mux/695
  "IW{2,1}(695,:)'"/1 -> dotprod695/1
  dotprod694/1 -> Mux/694
  "IW{2,1}(694,:)'"/1 -> dotprod694/1
  dotprod693/1 -> Mux/693
  "IW{2,1}(693,:)'"/1 -> dotprod693/1
  dotprod692/1 -> Mux/692
  "IW{2,1}(692,:)'"/1 -> dotprod692/1
  dotprod691/1 -> Mux/691
  "IW{2,1}(691,:)'"/1 -> dotprod691/1
  dotprod690/1 -> Mux/690
  "IW{2,1}(690,:)'"/1 -> dotprod690/1
  dotprod689/1 -> Mux/689
  "IW{2,1}(689,:)'"/1 -> dotprod689/1
  dotprod688/1 -> Mux/688
  "IW{2,1}(688,:)'"/1 -> dotprod688/1
  dotprod687/1 -> Mux/687
  "IW{2,1}(687,:)'"/1 -> dotprod687/1
  dotprod686/1 -> Mux/686
  "IW{2,1}(686,:)'"/1 -> dotprod686/1
  dotprod685/1 -> Mux/685
  "IW{2,1}(685,:)'"/1 -> dotprod685/1
  dotprod684/1 -> Mux/684
  "IW{2,1}(684,:)'"/1 -> dotprod684/1
  dotprod683/1 -> Mux/683
  "IW{2,1}(683,:)'"/1 -> dotprod683/1
  dotprod682/1 -> Mux/682
  "IW{2,1}(682,:)'"/1 -> dotprod682/1
  dotprod681/1 -> Mux/681
  "IW{2,1}(681,:)'"/1 -> dotprod681/1
  dotprod680/1 -> Mux/680
  "IW{2,1}(680,:)'"/1 -> dotprod680/1
  dotprod679/1 -> Mux/679
  "IW{2,1}(679,:)'"/1 -> dotprod679/1
  dotprod678/1 -> Mux/678
  "IW{2,1}(678,:)'"/1 -> dotprod678/1
  dotprod677/1 -> Mux/677
  "IW{2,1}(677,:)'"/1 -> dotprod677/1
  dotprod676/1 -> Mux/676
  "IW{2,1}(676,:)'"/1 -> dotprod676/1
  dotprod675/1 -> Mux/675
  "IW{2,1}(675,:)'"/1 -> dotprod675/1
  dotprod674/1 -> Mux/674
  "IW{2,1}(674,:)'"/1 -> dotprod674/1
  dotprod673/1 -> Mux/673
  "IW{2,1}(673,:)'"/1 -> dotprod673/1
  dotprod672/1 -> Mux/672
  "IW{2,1}(672,:)'"/1 -> dotprod672/1
  dotprod671/1 -> Mux/671
  "IW{2,1}(671,:)'"/1 -> dotprod671/1
  dotprod670/1 -> Mux/670
  "IW{2,1}(670,:)'"/1 -> dotprod670/1
  dotprod669/1 -> Mux/669
  "IW{2,1}(669,:)'"/1 -> dotprod669/1
  dotprod668/1 -> Mux/668
  "IW{2,1}(668,:)'"/1 -> dotprod668/1
  dotprod667/1 -> Mux/667
  "IW{2,1}(667,:)'"/1 -> dotprod667/1
  dotprod666/1 -> Mux/666
  "IW{2,1}(666,:)'"/1 -> dotprod666/1
  dotprod665/1 -> Mux/665
  "IW{2,1}(665,:)'"/1 -> dotprod665/1
  dotprod664/1 -> Mux/664
  "IW{2,1}(664,:)'"/1 -> dotprod664/1
  dotprod663/1 -> Mux/663
  "IW{2,1}(663,:)'"/1 -> dotprod663/1
  dotprod662/1 -> Mux/662
  "IW{2,1}(662,:)'"/1 -> dotprod662/1
  dotprod661/1 -> Mux/661
  "IW{2,1}(661,:)'"/1 -> dotprod661/1
  dotprod660/1 -> Mux/660
  "IW{2,1}(660,:)'"/1 -> dotprod660/1
  dotprod659/1 -> Mux/659
  "IW{2,1}(659,:)'"/1 -> dotprod659/1
  dotprod658/1 -> Mux/658
  "IW{2,1}(658,:)'"/1 -> dotprod658/1
  dotprod657/1 -> Mux/657
  "IW{2,1}(657,:)'"/1 -> dotprod657/1
  dotprod656/1 -> Mux/656
  "IW{2,1}(656,:)'"/1 -> dotprod656/1
  dotprod655/1 -> Mux/655
  "IW{2,1}(655,:)'"/1 -> dotprod655/1
  dotprod654/1 -> Mux/654
  "IW{2,1}(654,:)'"/1 -> dotprod654/1
  dotprod653/1 -> Mux/653
  "IW{2,1}(653,:)'"/1 -> dotprod653/1
  dotprod652/1 -> Mux/652
  "IW{2,1}(652,:)'"/1 -> dotprod652/1
  dotprod651/1 -> Mux/651
  "IW{2,1}(651,:)'"/1 -> dotprod651/1
  dotprod650/1 -> Mux/650
  "IW{2,1}(650,:)'"/1 -> dotprod650/1
  dotprod649/1 -> Mux/649
  "IW{2,1}(649,:)'"/1 -> dotprod649/1
  dotprod648/1 -> Mux/648
  "IW{2,1}(648,:)'"/1 -> dotprod648/1
  dotprod647/1 -> Mux/647
  "IW{2,1}(647,:)'"/1 -> dotprod647/1
  dotprod646/1 -> Mux/646
  "IW{2,1}(646,:)'"/1 -> dotprod646/1
  dotprod645/1 -> Mux/645
  "IW{2,1}(645,:)'"/1 -> dotprod645/1
  dotprod644/1 -> Mux/644
  "IW{2,1}(644,:)'"/1 -> dotprod644/1
  dotprod643/1 -> Mux/643
  "IW{2,1}(643,:)'"/1 -> dotprod643/1
  dotprod642/1 -> Mux/642
  "IW{2,1}(642,:)'"/1 -> dotprod642/1
  dotprod641/1 -> Mux/641
  "IW{2,1}(641,:)'"/1 -> dotprod641/1
  dotprod640/1 -> Mux/640
  "IW{2,1}(640,:)'"/1 -> dotprod640/1
  dotprod639/1 -> Mux/639
  "IW{2,1}(639,:)'"/1 -> dotprod639/1
  dotprod638/1 -> Mux/638
  "IW{2,1}(638,:)'"/1 -> dotprod638/1
  dotprod637/1 -> Mux/637
  "IW{2,1}(637,:)'"/1 -> dotprod637/1
  dotprod636/1 -> Mux/636
  "IW{2,1}(636,:)'"/1 -> dotprod636/1
  dotprod635/1 -> Mux/635
  "IW{2,1}(635,:)'"/1 -> dotprod635/1
  dotprod634/1 -> Mux/634
  "IW{2,1}(634,:)'"/1 -> dotprod634/1
  dotprod633/1 -> Mux/633
  "IW{2,1}(633,:)'"/1 -> dotprod633/1
  dotprod632/1 -> Mux/632
  "IW{2,1}(632,:)'"/1 -> dotprod632/1
  dotprod631/1 -> Mux/631
  "IW{2,1}(631,:)'"/1 -> dotprod631/1
  dotprod630/1 -> Mux/630
  "IW{2,1}(630,:)'"/1 -> dotprod630/1
  dotprod629/1 -> Mux/629
  "IW{2,1}(629,:)'"/1 -> dotprod629/1
  dotprod628/1 -> Mux/628
  "IW{2,1}(628,:)'"/1 -> dotprod628/1
  dotprod627/1 -> Mux/627
  "IW{2,1}(627,:)'"/1 -> dotprod627/1
  dotprod626/1 -> Mux/626
  "IW{2,1}(626,:)'"/1 -> dotprod626/1
  dotprod625/1 -> Mux/625
  "IW{2,1}(625,:)'"/1 -> dotprod625/1
  dotprod624/1 -> Mux/624
  "IW{2,1}(624,:)'"/1 -> dotprod624/1
  dotprod623/1 -> Mux/623
  "IW{2,1}(623,:)'"/1 -> dotprod623/1
  dotprod622/1 -> Mux/622
  "IW{2,1}(622,:)'"/1 -> dotprod622/1
  dotprod621/1 -> Mux/621
  "IW{2,1}(621,:)'"/1 -> dotprod621/1
  dotprod620/1 -> Mux/620
  "IW{2,1}(620,:)'"/1 -> dotprod620/1
  dotprod619/1 -> Mux/619
  "IW{2,1}(619,:)'"/1 -> dotprod619/1
  dotprod618/1 -> Mux/618
  "IW{2,1}(618,:)'"/1 -> dotprod618/1
  dotprod617/1 -> Mux/617
  "IW{2,1}(617,:)'"/1 -> dotprod617/1
  dotprod616/1 -> Mux/616
  "IW{2,1}(616,:)'"/1 -> dotprod616/1
  dotprod615/1 -> Mux/615
  "IW{2,1}(615,:)'"/1 -> dotprod615/1
  dotprod614/1 -> Mux/614
  "IW{2,1}(614,:)'"/1 -> dotprod614/1
  dotprod613/1 -> Mux/613
  "IW{2,1}(613,:)'"/1 -> dotprod613/1
  dotprod612/1 -> Mux/612
  "IW{2,1}(612,:)'"/1 -> dotprod612/1
  dotprod611/1 -> Mux/611
  "IW{2,1}(611,:)'"/1 -> dotprod611/1
  dotprod610/1 -> Mux/610
  "IW{2,1}(610,:)'"/1 -> dotprod610/1
  dotprod609/1 -> Mux/609
  "IW{2,1}(609,:)'"/1 -> dotprod609/1
  dotprod608/1 -> Mux/608
  "IW{2,1}(608,:)'"/1 -> dotprod608/1
  dotprod607/1 -> Mux/607
  "IW{2,1}(607,:)'"/1 -> dotprod607/1
  dotprod606/1 -> Mux/606
  "IW{2,1}(606,:)'"/1 -> dotprod606/1
  dotprod605/1 -> Mux/605
  "IW{2,1}(605,:)'"/1 -> dotprod605/1
  dotprod604/1 -> Mux/604
  "IW{2,1}(604,:)'"/1 -> dotprod604/1
  dotprod603/1 -> Mux/603
  "IW{2,1}(603,:)'"/1 -> dotprod603/1
  dotprod602/1 -> Mux/602
  "IW{2,1}(602,:)'"/1 -> dotprod602/1
  dotprod601/1 -> Mux/601
  "IW{2,1}(601,:)'"/1 -> dotprod601/1
  dotprod600/1 -> Mux/600
  "IW{2,1}(600,:)'"/1 -> dotprod600/1
  dotprod599/1 -> Mux/599
  "IW{2,1}(599,:)'"/1 -> dotprod599/1
  dotprod598/1 -> Mux/598
  "IW{2,1}(598,:)'"/1 -> dotprod598/1
  dotprod597/1 -> Mux/597
  "IW{2,1}(597,:)'"/1 -> dotprod597/1
  dotprod596/1 -> Mux/596
  "IW{2,1}(596,:)'"/1 -> dotprod596/1
  dotprod595/1 -> Mux/595
  "IW{2,1}(595,:)'"/1 -> dotprod595/1
  dotprod594/1 -> Mux/594
  "IW{2,1}(594,:)'"/1 -> dotprod594/1
  dotprod593/1 -> Mux/593
  "IW{2,1}(593,:)'"/1 -> dotprod593/1
  dotprod592/1 -> Mux/592
  "IW{2,1}(592,:)'"/1 -> dotprod592/1
  dotprod591/1 -> Mux/591
  "IW{2,1}(591,:)'"/1 -> dotprod591/1
  dotprod590/1 -> Mux/590
  "IW{2,1}(590,:)'"/1 -> dotprod590/1
  dotprod589/1 -> Mux/589
  "IW{2,1}(589,:)'"/1 -> dotprod589/1
  dotprod588/1 -> Mux/588
  "IW{2,1}(588,:)'"/1 -> dotprod588/1
  dotprod587/1 -> Mux/587
  "IW{2,1}(587,:)'"/1 -> dotprod587/1
  dotprod586/1 -> Mux/586
  "IW{2,1}(586,:)'"/1 -> dotprod586/1
  dotprod585/1 -> Mux/585
  "IW{2,1}(585,:)'"/1 -> dotprod585/1
  dotprod584/1 -> Mux/584
  "IW{2,1}(584,:)'"/1 -> dotprod584/1
  dotprod583/1 -> Mux/583
  "IW{2,1}(583,:)'"/1 -> dotprod583/1
  dotprod582/1 -> Mux/582
  "IW{2,1}(582,:)'"/1 -> dotprod582/1
  dotprod581/1 -> Mux/581
  "IW{2,1}(581,:)'"/1 -> dotprod581/1
  dotprod580/1 -> Mux/580
  "IW{2,1}(580,:)'"/1 -> dotprod580/1
  dotprod579/1 -> Mux/579
  "IW{2,1}(579,:)'"/1 -> dotprod579/1
  dotprod578/1 -> Mux/578
  "IW{2,1}(578,:)'"/1 -> dotprod578/1
  dotprod577/1 -> Mux/577
  "IW{2,1}(577,:)'"/1 -> dotprod577/1
  dotprod576/1 -> Mux/576
  "IW{2,1}(576,:)'"/1 -> dotprod576/1
  dotprod575/1 -> Mux/575
  "IW{2,1}(575,:)'"/1 -> dotprod575/1
  dotprod574/1 -> Mux/574
  "IW{2,1}(574,:)'"/1 -> dotprod574/1
  dotprod573/1 -> Mux/573
  "IW{2,1}(573,:)'"/1 -> dotprod573/1
  dotprod572/1 -> Mux/572
  "IW{2,1}(572,:)'"/1 -> dotprod572/1
  dotprod571/1 -> Mux/571
  "IW{2,1}(571,:)'"/1 -> dotprod571/1
  dotprod570/1 -> Mux/570
  "IW{2,1}(570,:)'"/1 -> dotprod570/1
  dotprod569/1 -> Mux/569
  "IW{2,1}(569,:)'"/1 -> dotprod569/1
  dotprod568/1 -> Mux/568
  "IW{2,1}(568,:)'"/1 -> dotprod568/1
  dotprod567/1 -> Mux/567
  "IW{2,1}(567,:)'"/1 -> dotprod567/1
  dotprod566/1 -> Mux/566
  "IW{2,1}(566,:)'"/1 -> dotprod566/1
  dotprod565/1 -> Mux/565
  "IW{2,1}(565,:)'"/1 -> dotprod565/1
  dotprod564/1 -> Mux/564
  "IW{2,1}(564,:)'"/1 -> dotprod564/1
  dotprod563/1 -> Mux/563
  "IW{2,1}(563,:)'"/1 -> dotprod563/1
  dotprod562/1 -> Mux/562
  "IW{2,1}(562,:)'"/1 -> dotprod562/1
  dotprod561/1 -> Mux/561
  "IW{2,1}(561,:)'"/1 -> dotprod561/1
  dotprod560/1 -> Mux/560
  "IW{2,1}(560,:)'"/1 -> dotprod560/1
  dotprod559/1 -> Mux/559
  "IW{2,1}(559,:)'"/1 -> dotprod559/1
  dotprod558/1 -> Mux/558
  "IW{2,1}(558,:)'"/1 -> dotprod558/1
  dotprod557/1 -> Mux/557
  "IW{2,1}(557,:)'"/1 -> dotprod557/1
  dotprod556/1 -> Mux/556
  "IW{2,1}(556,:)'"/1 -> dotprod556/1
  dotprod555/1 -> Mux/555
  "IW{2,1}(555,:)'"/1 -> dotprod555/1
  dotprod554/1 -> Mux/554
  "IW{2,1}(554,:)'"/1 -> dotprod554/1
  dotprod553/1 -> Mux/553
  "IW{2,1}(553,:)'"/1 -> dotprod553/1
  dotprod552/1 -> Mux/552
  "IW{2,1}(552,:)'"/1 -> dotprod552/1
  dotprod551/1 -> Mux/551
  "IW{2,1}(551,:)'"/1 -> dotprod551/1
  dotprod550/1 -> Mux/550
  "IW{2,1}(550,:)'"/1 -> dotprod550/1
  dotprod549/1 -> Mux/549
  "IW{2,1}(549,:)'"/1 -> dotprod549/1
  dotprod548/1 -> Mux/548
  "IW{2,1}(548,:)'"/1 -> dotprod548/1
  dotprod547/1 -> Mux/547
  "IW{2,1}(547,:)'"/1 -> dotprod547/1
  dotprod546/1 -> Mux/546
  "IW{2,1}(546,:)'"/1 -> dotprod546/1
  dotprod545/1 -> Mux/545
  "IW{2,1}(545,:)'"/1 -> dotprod545/1
  dotprod544/1 -> Mux/544
  "IW{2,1}(544,:)'"/1 -> dotprod544/1
  dotprod543/1 -> Mux/543
  "IW{2,1}(543,:)'"/1 -> dotprod543/1
  dotprod542/1 -> Mux/542
  "IW{2,1}(542,:)'"/1 -> dotprod542/1
  dotprod541/1 -> Mux/541
  "IW{2,1}(541,:)'"/1 -> dotprod541/1
  dotprod540/1 -> Mux/540
  "IW{2,1}(540,:)'"/1 -> dotprod540/1
  dotprod539/1 -> Mux/539
  "IW{2,1}(539,:)'"/1 -> dotprod539/1
  dotprod538/1 -> Mux/538
  "IW{2,1}(538,:)'"/1 -> dotprod538/1
  dotprod537/1 -> Mux/537
  "IW{2,1}(537,:)'"/1 -> dotprod537/1
  dotprod536/1 -> Mux/536
  "IW{2,1}(536,:)'"/1 -> dotprod536/1
  dotprod535/1 -> Mux/535
  "IW{2,1}(535,:)'"/1 -> dotprod535/1
  dotprod534/1 -> Mux/534
  "IW{2,1}(534,:)'"/1 -> dotprod534/1
  dotprod533/1 -> Mux/533
  "IW{2,1}(533,:)'"/1 -> dotprod533/1
  dotprod532/1 -> Mux/532
  "IW{2,1}(532,:)'"/1 -> dotprod532/1
  dotprod531/1 -> Mux/531
  "IW{2,1}(531,:)'"/1 -> dotprod531/1
  dotprod530/1 -> Mux/530
  "IW{2,1}(530,:)'"/1 -> dotprod530/1
  dotprod529/1 -> Mux/529
  "IW{2,1}(529,:)'"/1 -> dotprod529/1
  dotprod528/1 -> Mux/528
  "IW{2,1}(528,:)'"/1 -> dotprod528/1
  dotprod527/1 -> Mux/527
  "IW{2,1}(527,:)'"/1 -> dotprod527/1
  dotprod526/1 -> Mux/526
  "IW{2,1}(526,:)'"/1 -> dotprod526/1
  dotprod525/1 -> Mux/525
  "IW{2,1}(525,:)'"/1 -> dotprod525/1
  dotprod524/1 -> Mux/524
  "IW{2,1}(524,:)'"/1 -> dotprod524/1
  dotprod523/1 -> Mux/523
  "IW{2,1}(523,:)'"/1 -> dotprod523/1
  dotprod522/1 -> Mux/522
  "IW{2,1}(522,:)'"/1 -> dotprod522/1
  dotprod521/1 -> Mux/521
  "IW{2,1}(521,:)'"/1 -> dotprod521/1
  dotprod520/1 -> Mux/520
  "IW{2,1}(520,:)'"/1 -> dotprod520/1
  dotprod519/1 -> Mux/519
  "IW{2,1}(519,:)'"/1 -> dotprod519/1
  dotprod518/1 -> Mux/518
  "IW{2,1}(518,:)'"/1 -> dotprod518/1
  dotprod517/1 -> Mux/517
  "IW{2,1}(517,:)'"/1 -> dotprod517/1
  dotprod516/1 -> Mux/516
  "IW{2,1}(516,:)'"/1 -> dotprod516/1
  dotprod515/1 -> Mux/515
  "IW{2,1}(515,:)'"/1 -> dotprod515/1
  dotprod514/1 -> Mux/514
  "IW{2,1}(514,:)'"/1 -> dotprod514/1
  dotprod513/1 -> Mux/513
  "IW{2,1}(513,:)'"/1 -> dotprod513/1
  dotprod512/1 -> Mux/512
  "IW{2,1}(512,:)'"/1 -> dotprod512/1
  dotprod511/1 -> Mux/511
  "IW{2,1}(511,:)'"/1 -> dotprod511/1
  dotprod510/1 -> Mux/510
  "IW{2,1}(510,:)'"/1 -> dotprod510/1
  dotprod509/1 -> Mux/509
  "IW{2,1}(509,:)'"/1 -> dotprod509/1
  dotprod508/1 -> Mux/508
  "IW{2,1}(508,:)'"/1 -> dotprod508/1
  dotprod507/1 -> Mux/507
  "IW{2,1}(507,:)'"/1 -> dotprod507/1
  dotprod506/1 -> Mux/506
  "IW{2,1}(506,:)'"/1 -> dotprod506/1
  dotprod505/1 -> Mux/505
  "IW{2,1}(505,:)'"/1 -> dotprod505/1
  dotprod504/1 -> Mux/504
  "IW{2,1}(504,:)'"/1 -> dotprod504/1
  dotprod503/1 -> Mux/503
  "IW{2,1}(503,:)'"/1 -> dotprod503/1
  dotprod502/1 -> Mux/502
  "IW{2,1}(502,:)'"/1 -> dotprod502/1
  dotprod501/1 -> Mux/501
  "IW{2,1}(501,:)'"/1 -> dotprod501/1
  dotprod500/1 -> Mux/500
  "IW{2,1}(500,:)'"/1 -> dotprod500/1
  dotprod499/1 -> Mux/499
  "IW{2,1}(499,:)'"/1 -> dotprod499/1
  dotprod498/1 -> Mux/498
  "IW{2,1}(498,:)'"/1 -> dotprod498/1
  dotprod497/1 -> Mux/497
  "IW{2,1}(497,:)'"/1 -> dotprod497/1
  dotprod496/1 -> Mux/496
  "IW{2,1}(496,:)'"/1 -> dotprod496/1
  dotprod495/1 -> Mux/495
  "IW{2,1}(495,:)'"/1 -> dotprod495/1
  dotprod494/1 -> Mux/494
  "IW{2,1}(494,:)'"/1 -> dotprod494/1
  dotprod493/1 -> Mux/493
  "IW{2,1}(493,:)'"/1 -> dotprod493/1
  dotprod492/1 -> Mux/492
  "IW{2,1}(492,:)'"/1 -> dotprod492/1
  dotprod491/1 -> Mux/491
  "IW{2,1}(491,:)'"/1 -> dotprod491/1
  dotprod490/1 -> Mux/490
  "IW{2,1}(490,:)'"/1 -> dotprod490/1
  dotprod489/1 -> Mux/489
  "IW{2,1}(489,:)'"/1 -> dotprod489/1
  dotprod488/1 -> Mux/488
  "IW{2,1}(488,:)'"/1 -> dotprod488/1
  dotprod487/1 -> Mux/487
  "IW{2,1}(487,:)'"/1 -> dotprod487/1
  dotprod486/1 -> Mux/486
  "IW{2,1}(486,:)'"/1 -> dotprod486/1
  dotprod485/1 -> Mux/485
  "IW{2,1}(485,:)'"/1 -> dotprod485/1
  dotprod484/1 -> Mux/484
  "IW{2,1}(484,:)'"/1 -> dotprod484/1
  dotprod483/1 -> Mux/483
  "IW{2,1}(483,:)'"/1 -> dotprod483/1
  dotprod482/1 -> Mux/482
  "IW{2,1}(482,:)'"/1 -> dotprod482/1
  dotprod481/1 -> Mux/481
  "IW{2,1}(481,:)'"/1 -> dotprod481/1
  dotprod480/1 -> Mux/480
  "IW{2,1}(480,:)'"/1 -> dotprod480/1
  dotprod479/1 -> Mux/479
  "IW{2,1}(479,:)'"/1 -> dotprod479/1
  dotprod478/1 -> Mux/478
  "IW{2,1}(478,:)'"/1 -> dotprod478/1
  dotprod477/1 -> Mux/477
  "IW{2,1}(477,:)'"/1 -> dotprod477/1
  dotprod476/1 -> Mux/476
  "IW{2,1}(476,:)'"/1 -> dotprod476/1
  dotprod475/1 -> Mux/475
  "IW{2,1}(475,:)'"/1 -> dotprod475/1
  dotprod474/1 -> Mux/474
  "IW{2,1}(474,:)'"/1 -> dotprod474/1
  dotprod473/1 -> Mux/473
  "IW{2,1}(473,:)'"/1 -> dotprod473/1
  dotprod472/1 -> Mux/472
  "IW{2,1}(472,:)'"/1 -> dotprod472/1
  dotprod471/1 -> Mux/471
  "IW{2,1}(471,:)'"/1 -> dotprod471/1
  dotprod470/1 -> Mux/470
  "IW{2,1}(470,:)'"/1 -> dotprod470/1
  dotprod469/1 -> Mux/469
  "IW{2,1}(469,:)'"/1 -> dotprod469/1
  dotprod468/1 -> Mux/468
  "IW{2,1}(468,:)'"/1 -> dotprod468/1
  dotprod467/1 -> Mux/467
  "IW{2,1}(467,:)'"/1 -> dotprod467/1
  dotprod466/1 -> Mux/466
  "IW{2,1}(466,:)'"/1 -> dotprod466/1
  dotprod465/1 -> Mux/465
  "IW{2,1}(465,:)'"/1 -> dotprod465/1
  dotprod464/1 -> Mux/464
  "IW{2,1}(464,:)'"/1 -> dotprod464/1
  dotprod463/1 -> Mux/463
  "IW{2,1}(463,:)'"/1 -> dotprod463/1
  dotprod462/1 -> Mux/462
  "IW{2,1}(462,:)'"/1 -> dotprod462/1
  dotprod461/1 -> Mux/461
  "IW{2,1}(461,:)'"/1 -> dotprod461/1
  dotprod460/1 -> Mux/460
  "IW{2,1}(460,:)'"/1 -> dotprod460/1
  dotprod459/1 -> Mux/459
  "IW{2,1}(459,:)'"/1 -> dotprod459/1
  dotprod458/1 -> Mux/458
  "IW{2,1}(458,:)'"/1 -> dotprod458/1
  dotprod457/1 -> Mux/457
  "IW{2,1}(457,:)'"/1 -> dotprod457/1
  dotprod456/1 -> Mux/456
  "IW{2,1}(456,:)'"/1 -> dotprod456/1
  dotprod455/1 -> Mux/455
  "IW{2,1}(455,:)'"/1 -> dotprod455/1
  dotprod454/1 -> Mux/454
  "IW{2,1}(454,:)'"/1 -> dotprod454/1
  dotprod453/1 -> Mux/453
  "IW{2,1}(453,:)'"/1 -> dotprod453/1
  dotprod452/1 -> Mux/452
  "IW{2,1}(452,:)'"/1 -> dotprod452/1
  dotprod451/1 -> Mux/451
  "IW{2,1}(451,:)'"/1 -> dotprod451/1
  dotprod450/1 -> Mux/450
  "IW{2,1}(450,:)'"/1 -> dotprod450/1
  dotprod449/1 -> Mux/449
  "IW{2,1}(449,:)'"/1 -> dotprod449/1
  dotprod448/1 -> Mux/448
  "IW{2,1}(448,:)'"/1 -> dotprod448/1
  dotprod447/1 -> Mux/447
  "IW{2,1}(447,:)'"/1 -> dotprod447/1
  dotprod446/1 -> Mux/446
  "IW{2,1}(446,:)'"/1 -> dotprod446/1
  dotprod445/1 -> Mux/445
  "IW{2,1}(445,:)'"/1 -> dotprod445/1
  dotprod444/1 -> Mux/444
  "IW{2,1}(444,:)'"/1 -> dotprod444/1
  dotprod443/1 -> Mux/443
  "IW{2,1}(443,:)'"/1 -> dotprod443/1
  dotprod442/1 -> Mux/442
  "IW{2,1}(442,:)'"/1 -> dotprod442/1
  dotprod441/1 -> Mux/441
  "IW{2,1}(441,:)'"/1 -> dotprod441/1
  dotprod440/1 -> Mux/440
  "IW{2,1}(440,:)'"/1 -> dotprod440/1
  dotprod439/1 -> Mux/439
  "IW{2,1}(439,:)'"/1 -> dotprod439/1
  dotprod438/1 -> Mux/438
  "IW{2,1}(438,:)'"/1 -> dotprod438/1
  dotprod437/1 -> Mux/437
  "IW{2,1}(437,:)'"/1 -> dotprod437/1
  dotprod436/1 -> Mux/436
  "IW{2,1}(436,:)'"/1 -> dotprod436/1
  dotprod435/1 -> Mux/435
  "IW{2,1}(435,:)'"/1 -> dotprod435/1
  dotprod434/1 -> Mux/434
  "IW{2,1}(434,:)'"/1 -> dotprod434/1
  dotprod433/1 -> Mux/433
  "IW{2,1}(433,:)'"/1 -> dotprod433/1
  dotprod432/1 -> Mux/432
  "IW{2,1}(432,:)'"/1 -> dotprod432/1
  dotprod431/1 -> Mux/431
  "IW{2,1}(431,:)'"/1 -> dotprod431/1
  dotprod430/1 -> Mux/430
  "IW{2,1}(430,:)'"/1 -> dotprod430/1
  dotprod429/1 -> Mux/429
  "IW{2,1}(429,:)'"/1 -> dotprod429/1
  dotprod428/1 -> Mux/428
  "IW{2,1}(428,:)'"/1 -> dotprod428/1
  dotprod427/1 -> Mux/427
  "IW{2,1}(427,:)'"/1 -> dotprod427/1
  dotprod426/1 -> Mux/426
  "IW{2,1}(426,:)'"/1 -> dotprod426/1
  dotprod425/1 -> Mux/425
  "IW{2,1}(425,:)'"/1 -> dotprod425/1
  dotprod424/1 -> Mux/424
  "IW{2,1}(424,:)'"/1 -> dotprod424/1
  dotprod423/1 -> Mux/423
  "IW{2,1}(423,:)'"/1 -> dotprod423/1
  dotprod422/1 -> Mux/422
  "IW{2,1}(422,:)'"/1 -> dotprod422/1
  dotprod421/1 -> Mux/421
  "IW{2,1}(421,:)'"/1 -> dotprod421/1
  dotprod420/1 -> Mux/420
  "IW{2,1}(420,:)'"/1 -> dotprod420/1
  dotprod419/1 -> Mux/419
  "IW{2,1}(419,:)'"/1 -> dotprod419/1
  dotprod418/1 -> Mux/418
  "IW{2,1}(418,:)'"/1 -> dotprod418/1
  dotprod417/1 -> Mux/417
  "IW{2,1}(417,:)'"/1 -> dotprod417/1
  dotprod416/1 -> Mux/416
  "IW{2,1}(416,:)'"/1 -> dotprod416/1
  dotprod415/1 -> Mux/415
  "IW{2,1}(415,:)'"/1 -> dotprod415/1
  dotprod414/1 -> Mux/414
  "IW{2,1}(414,:)'"/1 -> dotprod414/1
  dotprod413/1 -> Mux/413
  "IW{2,1}(413,:)'"/1 -> dotprod413/1
  dotprod412/1 -> Mux/412
  "IW{2,1}(412,:)'"/1 -> dotprod412/1
  dotprod411/1 -> Mux/411
  "IW{2,1}(411,:)'"/1 -> dotprod411/1
  dotprod410/1 -> Mux/410
  "IW{2,1}(410,:)'"/1 -> dotprod410/1
  dotprod409/1 -> Mux/409
  "IW{2,1}(409,:)'"/1 -> dotprod409/1
  dotprod408/1 -> Mux/408
  "IW{2,1}(408,:)'"/1 -> dotprod408/1
  dotprod407/1 -> Mux/407
  "IW{2,1}(407,:)'"/1 -> dotprod407/1
  dotprod406/1 -> Mux/406
  "IW{2,1}(406,:)'"/1 -> dotprod406/1
  dotprod405/1 -> Mux/405
  "IW{2,1}(405,:)'"/1 -> dotprod405/1
  dotprod404/1 -> Mux/404
  "IW{2,1}(404,:)'"/1 -> dotprod404/1
  dotprod403/1 -> Mux/403
  "IW{2,1}(403,:)'"/1 -> dotprod403/1
  dotprod402/1 -> Mux/402
  "IW{2,1}(402,:)'"/1 -> dotprod402/1
  dotprod401/1 -> Mux/401
  "IW{2,1}(401,:)'"/1 -> dotprod401/1
  dotprod400/1 -> Mux/400
  "IW{2,1}(400,:)'"/1 -> dotprod400/1
  dotprod399/1 -> Mux/399
  "IW{2,1}(399,:)'"/1 -> dotprod399/1
  dotprod398/1 -> Mux/398
  "IW{2,1}(398,:)'"/1 -> dotprod398/1
  dotprod397/1 -> Mux/397
  "IW{2,1}(397,:)'"/1 -> dotprod397/1
  dotprod396/1 -> Mux/396
  "IW{2,1}(396,:)'"/1 -> dotprod396/1
  dotprod395/1 -> Mux/395
  "IW{2,1}(395,:)'"/1 -> dotprod395/1
  dotprod394/1 -> Mux/394
  "IW{2,1}(394,:)'"/1 -> dotprod394/1
  dotprod393/1 -> Mux/393
  "IW{2,1}(393,:)'"/1 -> dotprod393/1
  dotprod392/1 -> Mux/392
  "IW{2,1}(392,:)'"/1 -> dotprod392/1
  dotprod391/1 -> Mux/391
  "IW{2,1}(391,:)'"/1 -> dotprod391/1
  dotprod390/1 -> Mux/390
  "IW{2,1}(390,:)'"/1 -> dotprod390/1
  dotprod389/1 -> Mux/389
  "IW{2,1}(389,:)'"/1 -> dotprod389/1
  dotprod388/1 -> Mux/388
  "IW{2,1}(388,:)'"/1 -> dotprod388/1
  dotprod387/1 -> Mux/387
  "IW{2,1}(387,:)'"/1 -> dotprod387/1
  dotprod386/1 -> Mux/386
  "IW{2,1}(386,:)'"/1 -> dotprod386/1
  dotprod385/1 -> Mux/385
  "IW{2,1}(385,:)'"/1 -> dotprod385/1
  dotprod384/1 -> Mux/384
  "IW{2,1}(384,:)'"/1 -> dotprod384/1
  dotprod383/1 -> Mux/383
  "IW{2,1}(383,:)'"/1 -> dotprod383/1
  dotprod382/1 -> Mux/382
  "IW{2,1}(382,:)'"/1 -> dotprod382/1
  dotprod381/1 -> Mux/381
  "IW{2,1}(381,:)'"/1 -> dotprod381/1
  dotprod380/1 -> Mux/380
  "IW{2,1}(380,:)'"/1 -> dotprod380/1
  dotprod379/1 -> Mux/379
  "IW{2,1}(379,:)'"/1 -> dotprod379/1
  dotprod378/1 -> Mux/378
  "IW{2,1}(378,:)'"/1 -> dotprod378/1
  dotprod377/1 -> Mux/377
  "IW{2,1}(377,:)'"/1 -> dotprod377/1
  dotprod376/1 -> Mux/376
  "IW{2,1}(376,:)'"/1 -> dotprod376/1
  dotprod375/1 -> Mux/375
  "IW{2,1}(375,:)'"/1 -> dotprod375/1
  dotprod374/1 -> Mux/374
  "IW{2,1}(374,:)'"/1 -> dotprod374/1
  dotprod373/1 -> Mux/373
  "IW{2,1}(373,:)'"/1 -> dotprod373/1
  dotprod372/1 -> Mux/372
  "IW{2,1}(372,:)'"/1 -> dotprod372/1
  dotprod371/1 -> Mux/371
  "IW{2,1}(371,:)'"/1 -> dotprod371/1
  dotprod370/1 -> Mux/370
  "IW{2,1}(370,:)'"/1 -> dotprod370/1
  dotprod369/1 -> Mux/369
  "IW{2,1}(369,:)'"/1 -> dotprod369/1
  dotprod368/1 -> Mux/368
  "IW{2,1}(368,:)'"/1 -> dotprod368/1
  dotprod367/1 -> Mux/367
  "IW{2,1}(367,:)'"/1 -> dotprod367/1
  dotprod366/1 -> Mux/366
  "IW{2,1}(366,:)'"/1 -> dotprod366/1
  dotprod365/1 -> Mux/365
  "IW{2,1}(365,:)'"/1 -> dotprod365/1
  dotprod364/1 -> Mux/364
  "IW{2,1}(364,:)'"/1 -> dotprod364/1
  dotprod363/1 -> Mux/363
  "IW{2,1}(363,:)'"/1 -> dotprod363/1
  dotprod362/1 -> Mux/362
  "IW{2,1}(362,:)'"/1 -> dotprod362/1
  dotprod361/1 -> Mux/361
  "IW{2,1}(361,:)'"/1 -> dotprod361/1
  dotprod360/1 -> Mux/360
  "IW{2,1}(360,:)'"/1 -> dotprod360/1
  dotprod359/1 -> Mux/359
  "IW{2,1}(359,:)'"/1 -> dotprod359/1
  dotprod358/1 -> Mux/358
  "IW{2,1}(358,:)'"/1 -> dotprod358/1
  dotprod357/1 -> Mux/357
  "IW{2,1}(357,:)'"/1 -> dotprod357/1
  dotprod356/1 -> Mux/356
  "IW{2,1}(356,:)'"/1 -> dotprod356/1
  dotprod355/1 -> Mux/355
  "IW{2,1}(355,:)'"/1 -> dotprod355/1
  dotprod354/1 -> Mux/354
  "IW{2,1}(354,:)'"/1 -> dotprod354/1
  dotprod353/1 -> Mux/353
  "IW{2,1}(353,:)'"/1 -> dotprod353/1
  dotprod352/1 -> Mux/352
  "IW{2,1}(352,:)'"/1 -> dotprod352/1
  dotprod351/1 -> Mux/351
  "IW{2,1}(351,:)'"/1 -> dotprod351/1
  dotprod350/1 -> Mux/350
  "IW{2,1}(350,:)'"/1 -> dotprod350/1
  dotprod349/1 -> Mux/349
  "IW{2,1}(349,:)'"/1 -> dotprod349/1
  dotprod348/1 -> Mux/348
  "IW{2,1}(348,:)'"/1 -> dotprod348/1
  dotprod347/1 -> Mux/347
  "IW{2,1}(347,:)'"/1 -> dotprod347/1
  dotprod346/1 -> Mux/346
  "IW{2,1}(346,:)'"/1 -> dotprod346/1
  dotprod345/1 -> Mux/345
  "IW{2,1}(345,:)'"/1 -> dotprod345/1
  dotprod344/1 -> Mux/344
  "IW{2,1}(344,:)'"/1 -> dotprod344/1
  dotprod343/1 -> Mux/343
  "IW{2,1}(343,:)'"/1 -> dotprod343/1
  dotprod342/1 -> Mux/342
  "IW{2,1}(342,:)'"/1 -> dotprod342/1
  dotprod341/1 -> Mux/341
  "IW{2,1}(341,:)'"/1 -> dotprod341/1
  dotprod340/1 -> Mux/340
  "IW{2,1}(340,:)'"/1 -> dotprod340/1
  dotprod339/1 -> Mux/339
  "IW{2,1}(339,:)'"/1 -> dotprod339/1
  dotprod338/1 -> Mux/338
  "IW{2,1}(338,:)'"/1 -> dotprod338/1
  dotprod337/1 -> Mux/337
  "IW{2,1}(337,:)'"/1 -> dotprod337/1
  dotprod336/1 -> Mux/336
  "IW{2,1}(336,:)'"/1 -> dotprod336/1
  dotprod335/1 -> Mux/335
  "IW{2,1}(335,:)'"/1 -> dotprod335/1
  dotprod334/1 -> Mux/334
  "IW{2,1}(334,:)'"/1 -> dotprod334/1
  dotprod333/1 -> Mux/333
  "IW{2,1}(333,:)'"/1 -> dotprod333/1
  dotprod332/1 -> Mux/332
  "IW{2,1}(332,:)'"/1 -> dotprod332/1
  dotprod331/1 -> Mux/331
  "IW{2,1}(331,:)'"/1 -> dotprod331/1
  dotprod330/1 -> Mux/330
  "IW{2,1}(330,:)'"/1 -> dotprod330/1
  dotprod329/1 -> Mux/329
  "IW{2,1}(329,:)'"/1 -> dotprod329/1
  dotprod328/1 -> Mux/328
  "IW{2,1}(328,:)'"/1 -> dotprod328/1
  dotprod327/1 -> Mux/327
  "IW{2,1}(327,:)'"/1 -> dotprod327/1
  dotprod326/1 -> Mux/326
  "IW{2,1}(326,:)'"/1 -> dotprod326/1
  dotprod325/1 -> Mux/325
  "IW{2,1}(325,:)'"/1 -> dotprod325/1
  dotprod324/1 -> Mux/324
  "IW{2,1}(324,:)'"/1 -> dotprod324/1
  dotprod323/1 -> Mux/323
  "IW{2,1}(323,:)'"/1 -> dotprod323/1
  dotprod322/1 -> Mux/322
  "IW{2,1}(322,:)'"/1 -> dotprod322/1
  dotprod321/1 -> Mux/321
  "IW{2,1}(321,:)'"/1 -> dotprod321/1
  dotprod320/1 -> Mux/320
  "IW{2,1}(320,:)'"/1 -> dotprod320/1
  dotprod319/1 -> Mux/319
  "IW{2,1}(319,:)'"/1 -> dotprod319/1
  dotprod318/1 -> Mux/318
  "IW{2,1}(318,:)'"/1 -> dotprod318/1
  dotprod317/1 -> Mux/317
  "IW{2,1}(317,:)'"/1 -> dotprod317/1
  dotprod316/1 -> Mux/316
  "IW{2,1}(316,:)'"/1 -> dotprod316/1
  dotprod315/1 -> Mux/315
  "IW{2,1}(315,:)'"/1 -> dotprod315/1
  dotprod314/1 -> Mux/314
  "IW{2,1}(314,:)'"/1 -> dotprod314/1
  dotprod313/1 -> Mux/313
  "IW{2,1}(313,:)'"/1 -> dotprod313/1
  dotprod312/1 -> Mux/312
  "IW{2,1}(312,:)'"/1 -> dotprod312/1
  dotprod311/1 -> Mux/311
  "IW{2,1}(311,:)'"/1 -> dotprod311/1
  dotprod310/1 -> Mux/310
  "IW{2,1}(310,:)'"/1 -> dotprod310/1
  dotprod309/1 -> Mux/309
  "IW{2,1}(309,:)'"/1 -> dotprod309/1
  dotprod308/1 -> Mux/308
  "IW{2,1}(308,:)'"/1 -> dotprod308/1
  dotprod307/1 -> Mux/307
  "IW{2,1}(307,:)'"/1 -> dotprod307/1
  dotprod306/1 -> Mux/306
  "IW{2,1}(306,:)'"/1 -> dotprod306/1
  dotprod305/1 -> Mux/305
  "IW{2,1}(305,:)'"/1 -> dotprod305/1
  dotprod304/1 -> Mux/304
  "IW{2,1}(304,:)'"/1 -> dotprod304/1
  dotprod303/1 -> Mux/303
  "IW{2,1}(303,:)'"/1 -> dotprod303/1
  dotprod302/1 -> Mux/302
  "IW{2,1}(302,:)'"/1 -> dotprod302/1
  dotprod301/1 -> Mux/301
  "IW{2,1}(301,:)'"/1 -> dotprod301/1
  dotprod300/1 -> Mux/300
  "IW{2,1}(300,:)'"/1 -> dotprod300/1
  dotprod299/1 -> Mux/299
  "IW{2,1}(299,:)'"/1 -> dotprod299/1
  dotprod298/1 -> Mux/298
  "IW{2,1}(298,:)'"/1 -> dotprod298/1
  dotprod297/1 -> Mux/297
  "IW{2,1}(297,:)'"/1 -> dotprod297/1
  dotprod296/1 -> Mux/296
  "IW{2,1}(296,:)'"/1 -> dotprod296/1
  dotprod295/1 -> Mux/295
  "IW{2,1}(295,:)'"/1 -> dotprod295/1
  dotprod294/1 -> Mux/294
  "IW{2,1}(294,:)'"/1 -> dotprod294/1
  dotprod293/1 -> Mux/293
  "IW{2,1}(293,:)'"/1 -> dotprod293/1
  dotprod292/1 -> Mux/292
  "IW{2,1}(292,:)'"/1 -> dotprod292/1
  dotprod291/1 -> Mux/291
  "IW{2,1}(291,:)'"/1 -> dotprod291/1
  dotprod290/1 -> Mux/290
  "IW{2,1}(290,:)'"/1 -> dotprod290/1
  dotprod289/1 -> Mux/289
  "IW{2,1}(289,:)'"/1 -> dotprod289/1
  dotprod288/1 -> Mux/288
  "IW{2,1}(288,:)'"/1 -> dotprod288/1
  dotprod287/1 -> Mux/287
  "IW{2,1}(287,:)'"/1 -> dotprod287/1
  dotprod286/1 -> Mux/286
  "IW{2,1}(286,:)'"/1 -> dotprod286/1
  dotprod285/1 -> Mux/285
  "IW{2,1}(285,:)'"/1 -> dotprod285/1
  dotprod284/1 -> Mux/284
  "IW{2,1}(284,:)'"/1 -> dotprod284/1
  dotprod283/1 -> Mux/283
  "IW{2,1}(283,:)'"/1 -> dotprod283/1
  dotprod282/1 -> Mux/282
  "IW{2,1}(282,:)'"/1 -> dotprod282/1
  dotprod281/1 -> Mux/281
  "IW{2,1}(281,:)'"/1 -> dotprod281/1
  dotprod280/1 -> Mux/280
  "IW{2,1}(280,:)'"/1 -> dotprod280/1
  dotprod279/1 -> Mux/279
  "IW{2,1}(279,:)'"/1 -> dotprod279/1
  dotprod278/1 -> Mux/278
  "IW{2,1}(278,:)'"/1 -> dotprod278/1
  dotprod277/1 -> Mux/277
  "IW{2,1}(277,:)'"/1 -> dotprod277/1
  dotprod276/1 -> Mux/276
  "IW{2,1}(276,:)'"/1 -> dotprod276/1
  dotprod275/1 -> Mux/275
  "IW{2,1}(275,:)'"/1 -> dotprod275/1
  dotprod274/1 -> Mux/274
  "IW{2,1}(274,:)'"/1 -> dotprod274/1
  dotprod273/1 -> Mux/273
  "IW{2,1}(273,:)'"/1 -> dotprod273/1
  dotprod272/1 -> Mux/272
  "IW{2,1}(272,:)'"/1 -> dotprod272/1
  dotprod271/1 -> Mux/271
  "IW{2,1}(271,:)'"/1 -> dotprod271/1
  dotprod270/1 -> Mux/270
  "IW{2,1}(270,:)'"/1 -> dotprod270/1
  dotprod269/1 -> Mux/269
  "IW{2,1}(269,:)'"/1 -> dotprod269/1
  dotprod268/1 -> Mux/268
  "IW{2,1}(268,:)'"/1 -> dotprod268/1
  dotprod267/1 -> Mux/267
  "IW{2,1}(267,:)'"/1 -> dotprod267/1
  dotprod266/1 -> Mux/266
  "IW{2,1}(266,:)'"/1 -> dotprod266/1
  dotprod265/1 -> Mux/265
  "IW{2,1}(265,:)'"/1 -> dotprod265/1
  dotprod264/1 -> Mux/264
  "IW{2,1}(264,:)'"/1 -> dotprod264/1
  dotprod263/1 -> Mux/263
  "IW{2,1}(263,:)'"/1 -> dotprod263/1
  dotprod262/1 -> Mux/262
  "IW{2,1}(262,:)'"/1 -> dotprod262/1
  dotprod261/1 -> Mux/261
  "IW{2,1}(261,:)'"/1 -> dotprod261/1
  dotprod260/1 -> Mux/260
  "IW{2,1}(260,:)'"/1 -> dotprod260/1
  dotprod259/1 -> Mux/259
  "IW{2,1}(259,:)'"/1 -> dotprod259/1
  dotprod258/1 -> Mux/258
  "IW{2,1}(258,:)'"/1 -> dotprod258/1
  dotprod257/1 -> Mux/257
  "IW{2,1}(257,:)'"/1 -> dotprod257/1
  dotprod256/1 -> Mux/256
  "IW{2,1}(256,:)'"/1 -> dotprod256/1
  dotprod255/1 -> Mux/255
  "IW{2,1}(255,:)'"/1 -> dotprod255/1
  dotprod254/1 -> Mux/254
  "IW{2,1}(254,:)'"/1 -> dotprod254/1
  dotprod253/1 -> Mux/253
  "IW{2,1}(253,:)'"/1 -> dotprod253/1
  dotprod252/1 -> Mux/252
  "IW{2,1}(252,:)'"/1 -> dotprod252/1
  dotprod251/1 -> Mux/251
  "IW{2,1}(251,:)'"/1 -> dotprod251/1
  dotprod250/1 -> Mux/250
  "IW{2,1}(250,:)'"/1 -> dotprod250/1
  dotprod249/1 -> Mux/249
  "IW{2,1}(249,:)'"/1 -> dotprod249/1
  dotprod248/1 -> Mux/248
  "IW{2,1}(248,:)'"/1 -> dotprod248/1
  dotprod247/1 -> Mux/247
  "IW{2,1}(247,:)'"/1 -> dotprod247/1
  dotprod246/1 -> Mux/246
  "IW{2,1}(246,:)'"/1 -> dotprod246/1
  dotprod245/1 -> Mux/245
  "IW{2,1}(245,:)'"/1 -> dotprod245/1
  dotprod244/1 -> Mux/244
  "IW{2,1}(244,:)'"/1 -> dotprod244/1
  dotprod243/1 -> Mux/243
  "IW{2,1}(243,:)'"/1 -> dotprod243/1
  dotprod242/1 -> Mux/242
  "IW{2,1}(242,:)'"/1 -> dotprod242/1
  dotprod241/1 -> Mux/241
  "IW{2,1}(241,:)'"/1 -> dotprod241/1
  dotprod240/1 -> Mux/240
  "IW{2,1}(240,:)'"/1 -> dotprod240/1
  dotprod239/1 -> Mux/239
  "IW{2,1}(239,:)'"/1 -> dotprod239/1
  dotprod238/1 -> Mux/238
  "IW{2,1}(238,:)'"/1 -> dotprod238/1
  dotprod237/1 -> Mux/237
  "IW{2,1}(237,:)'"/1 -> dotprod237/1
  dotprod236/1 -> Mux/236
  "IW{2,1}(236,:)'"/1 -> dotprod236/1
  dotprod235/1 -> Mux/235
  "IW{2,1}(235,:)'"/1 -> dotprod235/1
  dotprod234/1 -> Mux/234
  "IW{2,1}(234,:)'"/1 -> dotprod234/1
  dotprod233/1 -> Mux/233
  "IW{2,1}(233,:)'"/1 -> dotprod233/1
  dotprod232/1 -> Mux/232
  "IW{2,1}(232,:)'"/1 -> dotprod232/1
  dotprod231/1 -> Mux/231
  "IW{2,1}(231,:)'"/1 -> dotprod231/1
  dotprod230/1 -> Mux/230
  "IW{2,1}(230,:)'"/1 -> dotprod230/1
  dotprod229/1 -> Mux/229
  "IW{2,1}(229,:)'"/1 -> dotprod229/1
  dotprod228/1 -> Mux/228
  "IW{2,1}(228,:)'"/1 -> dotprod228/1
  dotprod227/1 -> Mux/227
  "IW{2,1}(227,:)'"/1 -> dotprod227/1
  dotprod226/1 -> Mux/226
  "IW{2,1}(226,:)'"/1 -> dotprod226/1
  dotprod225/1 -> Mux/225
  "IW{2,1}(225,:)'"/1 -> dotprod225/1
  dotprod224/1 -> Mux/224
  "IW{2,1}(224,:)'"/1 -> dotprod224/1
  dotprod223/1 -> Mux/223
  "IW{2,1}(223,:)'"/1 -> dotprod223/1
  dotprod222/1 -> Mux/222
  "IW{2,1}(222,:)'"/1 -> dotprod222/1
  dotprod221/1 -> Mux/221
  "IW{2,1}(221,:)'"/1 -> dotprod221/1
  dotprod220/1 -> Mux/220
  "IW{2,1}(220,:)'"/1 -> dotprod220/1
  dotprod219/1 -> Mux/219
  "IW{2,1}(219,:)'"/1 -> dotprod219/1
  dotprod218/1 -> Mux/218
  "IW{2,1}(218,:)'"/1 -> dotprod218/1
  dotprod217/1 -> Mux/217
  "IW{2,1}(217,:)'"/1 -> dotprod217/1
  dotprod216/1 -> Mux/216
  "IW{2,1}(216,:)'"/1 -> dotprod216/1
  dotprod215/1 -> Mux/215
  "IW{2,1}(215,:)'"/1 -> dotprod215/1
  dotprod214/1 -> Mux/214
  "IW{2,1}(214,:)'"/1 -> dotprod214/1
  dotprod213/1 -> Mux/213
  "IW{2,1}(213,:)'"/1 -> dotprod213/1
  dotprod212/1 -> Mux/212
  "IW{2,1}(212,:)'"/1 -> dotprod212/1
  dotprod211/1 -> Mux/211
  "IW{2,1}(211,:)'"/1 -> dotprod211/1
  dotprod210/1 -> Mux/210
  "IW{2,1}(210,:)'"/1 -> dotprod210/1
  dotprod209/1 -> Mux/209
  "IW{2,1}(209,:)'"/1 -> dotprod209/1
  dotprod208/1 -> Mux/208
  "IW{2,1}(208,:)'"/1 -> dotprod208/1
  dotprod207/1 -> Mux/207
  "IW{2,1}(207,:)'"/1 -> dotprod207/1
  dotprod206/1 -> Mux/206
  "IW{2,1}(206,:)'"/1 -> dotprod206/1
  dotprod205/1 -> Mux/205
  "IW{2,1}(205,:)'"/1 -> dotprod205/1
  dotprod204/1 -> Mux/204
  "IW{2,1}(204,:)'"/1 -> dotprod204/1
  dotprod203/1 -> Mux/203
  "IW{2,1}(203,:)'"/1 -> dotprod203/1
  dotprod202/1 -> Mux/202
  "IW{2,1}(202,:)'"/1 -> dotprod202/1
  dotprod201/1 -> Mux/201
  "IW{2,1}(201,:)'"/1 -> dotprod201/1
  dotprod200/1 -> Mux/200
  "IW{2,1}(200,:)'"/1 -> dotprod200/1
  dotprod199/1 -> Mux/199
  "IW{2,1}(199,:)'"/1 -> dotprod199/1
  dotprod198/1 -> Mux/198
  "IW{2,1}(198,:)'"/1 -> dotprod198/1
  dotprod197/1 -> Mux/197
  "IW{2,1}(197,:)'"/1 -> dotprod197/1
  dotprod196/1 -> Mux/196
  "IW{2,1}(196,:)'"/1 -> dotprod196/1
  dotprod195/1 -> Mux/195
  "IW{2,1}(195,:)'"/1 -> dotprod195/1
  dotprod194/1 -> Mux/194
  "IW{2,1}(194,:)'"/1 -> dotprod194/1
  dotprod193/1 -> Mux/193
  "IW{2,1}(193,:)'"/1 -> dotprod193/1
  dotprod192/1 -> Mux/192
  "IW{2,1}(192,:)'"/1 -> dotprod192/1
  dotprod191/1 -> Mux/191
  "IW{2,1}(191,:)'"/1 -> dotprod191/1
  dotprod190/1 -> Mux/190
  "IW{2,1}(190,:)'"/1 -> dotprod190/1
  dotprod189/1 -> Mux/189
  "IW{2,1}(189,:)'"/1 -> dotprod189/1
  dotprod188/1 -> Mux/188
  "IW{2,1}(188,:)'"/1 -> dotprod188/1
  dotprod187/1 -> Mux/187
  "IW{2,1}(187,:)'"/1 -> dotprod187/1
  dotprod186/1 -> Mux/186
  "IW{2,1}(186,:)'"/1 -> dotprod186/1
  dotprod185/1 -> Mux/185
  "IW{2,1}(185,:)'"/1 -> dotprod185/1
  dotprod184/1 -> Mux/184
  "IW{2,1}(184,:)'"/1 -> dotprod184/1
  dotprod183/1 -> Mux/183
  "IW{2,1}(183,:)'"/1 -> dotprod183/1
  dotprod182/1 -> Mux/182
  "IW{2,1}(182,:)'"/1 -> dotprod182/1
  dotprod181/1 -> Mux/181
  "IW{2,1}(181,:)'"/1 -> dotprod181/1
  dotprod180/1 -> Mux/180
  "IW{2,1}(180,:)'"/1 -> dotprod180/1
  dotprod179/1 -> Mux/179
  "IW{2,1}(179,:)'"/1 -> dotprod179/1
  dotprod178/1 -> Mux/178
  "IW{2,1}(178,:)'"/1 -> dotprod178/1
  dotprod177/1 -> Mux/177
  "IW{2,1}(177,:)'"/1 -> dotprod177/1
  dotprod176/1 -> Mux/176
  "IW{2,1}(176,:)'"/1 -> dotprod176/1
  dotprod175/1 -> Mux/175
  "IW{2,1}(175,:)'"/1 -> dotprod175/1
  dotprod174/1 -> Mux/174
  "IW{2,1}(174,:)'"/1 -> dotprod174/1
  dotprod173/1 -> Mux/173
  "IW{2,1}(173,:)'"/1 -> dotprod173/1
  dotprod172/1 -> Mux/172
  "IW{2,1}(172,:)'"/1 -> dotprod172/1
  dotprod171/1 -> Mux/171
  "IW{2,1}(171,:)'"/1 -> dotprod171/1
  dotprod170/1 -> Mux/170
  "IW{2,1}(170,:)'"/1 -> dotprod170/1
  dotprod169/1 -> Mux/169
  "IW{2,1}(169,:)'"/1 -> dotprod169/1
  dotprod168/1 -> Mux/168
  "IW{2,1}(168,:)'"/1 -> dotprod168/1
  dotprod167/1 -> Mux/167
  "IW{2,1}(167,:)'"/1 -> dotprod167/1
  dotprod166/1 -> Mux/166
  "IW{2,1}(166,:)'"/1 -> dotprod166/1
  dotprod165/1 -> Mux/165
  "IW{2,1}(165,:)'"/1 -> dotprod165/1
  dotprod164/1 -> Mux/164
  "IW{2,1}(164,:)'"/1 -> dotprod164/1
  dotprod163/1 -> Mux/163
  "IW{2,1}(163,:)'"/1 -> dotprod163/1
  dotprod162/1 -> Mux/162
  "IW{2,1}(162,:)'"/1 -> dotprod162/1
  dotprod161/1 -> Mux/161
  "IW{2,1}(161,:)'"/1 -> dotprod161/1
  dotprod160/1 -> Mux/160
  "IW{2,1}(160,:)'"/1 -> dotprod160/1
  dotprod159/1 -> Mux/159
  "IW{2,1}(159,:)'"/1 -> dotprod159/1
  dotprod158/1 -> Mux/158
  "IW{2,1}(158,:)'"/1 -> dotprod158/1
  dotprod157/1 -> Mux/157
  "IW{2,1}(157,:)'"/1 -> dotprod157/1
  dotprod156/1 -> Mux/156
  "IW{2,1}(156,:)'"/1 -> dotprod156/1
  dotprod155/1 -> Mux/155
  "IW{2,1}(155,:)'"/1 -> dotprod155/1
  dotprod154/1 -> Mux/154
  "IW{2,1}(154,:)'"/1 -> dotprod154/1
  dotprod153/1 -> Mux/153
  "IW{2,1}(153,:)'"/1 -> dotprod153/1
  dotprod152/1 -> Mux/152
  "IW{2,1}(152,:)'"/1 -> dotprod152/1
  dotprod151/1 -> Mux/151
  "IW{2,1}(151,:)'"/1 -> dotprod151/1
  dotprod150/1 -> Mux/150
  "IW{2,1}(150,:)'"/1 -> dotprod150/1
  dotprod149/1 -> Mux/149
  "IW{2,1}(149,:)'"/1 -> dotprod149/1
  dotprod148/1 -> Mux/148
  "IW{2,1}(148,:)'"/1 -> dotprod148/1
  dotprod147/1 -> Mux/147
  "IW{2,1}(147,:)'"/1 -> dotprod147/1
  dotprod146/1 -> Mux/146
  "IW{2,1}(146,:)'"/1 -> dotprod146/1
  dotprod145/1 -> Mux/145
  "IW{2,1}(145,:)'"/1 -> dotprod145/1
  dotprod144/1 -> Mux/144
  "IW{2,1}(144,:)'"/1 -> dotprod144/1
  dotprod143/1 -> Mux/143
  "IW{2,1}(143,:)'"/1 -> dotprod143/1
  dotprod142/1 -> Mux/142
  "IW{2,1}(142,:)'"/1 -> dotprod142/1
  dotprod141/1 -> Mux/141
  "IW{2,1}(141,:)'"/1 -> dotprod141/1
  dotprod140/1 -> Mux/140
  "IW{2,1}(140,:)'"/1 -> dotprod140/1
  dotprod139/1 -> Mux/139
  "IW{2,1}(139,:)'"/1 -> dotprod139/1
  dotprod138/1 -> Mux/138
  "IW{2,1}(138,:)'"/1 -> dotprod138/1
  dotprod137/1 -> Mux/137
  "IW{2,1}(137,:)'"/1 -> dotprod137/1
  dotprod136/1 -> Mux/136
  "IW{2,1}(136,:)'"/1 -> dotprod136/1
  dotprod135/1 -> Mux/135
  "IW{2,1}(135,:)'"/1 -> dotprod135/1
  dotprod134/1 -> Mux/134
  "IW{2,1}(134,:)'"/1 -> dotprod134/1
  dotprod133/1 -> Mux/133
  "IW{2,1}(133,:)'"/1 -> dotprod133/1
  dotprod132/1 -> Mux/132
  "IW{2,1}(132,:)'"/1 -> dotprod132/1
  dotprod131/1 -> Mux/131
  "IW{2,1}(131,:)'"/1 -> dotprod131/1
  dotprod130/1 -> Mux/130
  "IW{2,1}(130,:)'"/1 -> dotprod130/1
  dotprod129/1 -> Mux/129
  "IW{2,1}(129,:)'"/1 -> dotprod129/1
  dotprod128/1 -> Mux/128
  "IW{2,1}(128,:)'"/1 -> dotprod128/1
  dotprod127/1 -> Mux/127
  "IW{2,1}(127,:)'"/1 -> dotprod127/1
  dotprod126/1 -> Mux/126
  "IW{2,1}(126,:)'"/1 -> dotprod126/1
  dotprod125/1 -> Mux/125
  "IW{2,1}(125,:)'"/1 -> dotprod125/1
  dotprod124/1 -> Mux/124
  "IW{2,1}(124,:)'"/1 -> dotprod124/1
  dotprod123/1 -> Mux/123
  "IW{2,1}(123,:)'"/1 -> dotprod123/1
  dotprod122/1 -> Mux/122
  "IW{2,1}(122,:)'"/1 -> dotprod122/1
  dotprod121/1 -> Mux/121
  "IW{2,1}(121,:)'"/1 -> dotprod121/1
  dotprod120/1 -> Mux/120
  "IW{2,1}(120,:)'"/1 -> dotprod120/1
  dotprod119/1 -> Mux/119
  "IW{2,1}(119,:)'"/1 -> dotprod119/1
  dotprod118/1 -> Mux/118
  "IW{2,1}(118,:)'"/1 -> dotprod118/1
  dotprod117/1 -> Mux/117
  "IW{2,1}(117,:)'"/1 -> dotprod117/1
  dotprod116/1 -> Mux/116
  "IW{2,1}(116,:)'"/1 -> dotprod116/1
  dotprod115/1 -> Mux/115
  "IW{2,1}(115,:)'"/1 -> dotprod115/1
  dotprod114/1 -> Mux/114
  "IW{2,1}(114,:)'"/1 -> dotprod114/1
  dotprod113/1 -> Mux/113
  "IW{2,1}(113,:)'"/1 -> dotprod113/1
  dotprod112/1 -> Mux/112
  "IW{2,1}(112,:)'"/1 -> dotprod112/1
  dotprod111/1 -> Mux/111
  "IW{2,1}(111,:)'"/1 -> dotprod111/1
  dotprod110/1 -> Mux/110
  "IW{2,1}(110,:)'"/1 -> dotprod110/1
  dotprod109/1 -> Mux/109
  "IW{2,1}(109,:)'"/1 -> dotprod109/1
  dotprod108/1 -> Mux/108
  "IW{2,1}(108,:)'"/1 -> dotprod108/1
  dotprod107/1 -> Mux/107
  "IW{2,1}(107,:)'"/1 -> dotprod107/1
  dotprod106/1 -> Mux/106
  "IW{2,1}(106,:)'"/1 -> dotprod106/1
  dotprod105/1 -> Mux/105
  "IW{2,1}(105,:)'"/1 -> dotprod105/1
  dotprod104/1 -> Mux/104
  "IW{2,1}(104,:)'"/1 -> dotprod104/1
  dotprod103/1 -> Mux/103
  "IW{2,1}(103,:)'"/1 -> dotprod103/1
  dotprod102/1 -> Mux/102
  "IW{2,1}(102,:)'"/1 -> dotprod102/1
  dotprod101/1 -> Mux/101
  "IW{2,1}(101,:)'"/1 -> dotprod101/1
  dotprod100/1 -> Mux/100
  "IW{2,1}(100,:)'"/1 -> dotprod100/1
  dotprod99/1 -> Mux/99
  "IW{2,1}(99,:)'"/1 -> dotprod99/1
  dotprod98/1 -> Mux/98
  "IW{2,1}(98,:)'"/1 -> dotprod98/1
  dotprod97/1 -> Mux/97
  "IW{2,1}(97,:)'"/1 -> dotprod97/1
  dotprod96/1 -> Mux/96
  "IW{2,1}(96,:)'"/1 -> dotprod96/1
  dotprod95/1 -> Mux/95
  "IW{2,1}(95,:)'"/1 -> dotprod95/1
  dotprod94/1 -> Mux/94
  "IW{2,1}(94,:)'"/1 -> dotprod94/1
  dotprod93/1 -> Mux/93
  "IW{2,1}(93,:)'"/1 -> dotprod93/1
  dotprod92/1 -> Mux/92
  "IW{2,1}(92,:)'"/1 -> dotprod92/1
  dotprod91/1 -> Mux/91
  "IW{2,1}(91,:)'"/1 -> dotprod91/1
  dotprod90/1 -> Mux/90
  "IW{2,1}(90,:)'"/1 -> dotprod90/1
  dotprod89/1 -> Mux/89
  "IW{2,1}(89,:)'"/1 -> dotprod89/1
  dotprod88/1 -> Mux/88
  "IW{2,1}(88,:)'"/1 -> dotprod88/1
  dotprod87/1 -> Mux/87
  "IW{2,1}(87,:)'"/1 -> dotprod87/1
  dotprod86/1 -> Mux/86
  "IW{2,1}(86,:)'"/1 -> dotprod86/1
  dotprod85/1 -> Mux/85
  "IW{2,1}(85,:)'"/1 -> dotprod85/1
  dotprod84/1 -> Mux/84
  "IW{2,1}(84,:)'"/1 -> dotprod84/1
  dotprod83/1 -> Mux/83
  "IW{2,1}(83,:)'"/1 -> dotprod83/1
  dotprod82/1 -> Mux/82
  "IW{2,1}(82,:)'"/1 -> dotprod82/1
  dotprod81/1 -> Mux/81
  "IW{2,1}(81,:)'"/1 -> dotprod81/1
  dotprod80/1 -> Mux/80
  "IW{2,1}(80,:)'"/1 -> dotprod80/1
  dotprod79/1 -> Mux/79
  "IW{2,1}(79,:)'"/1 -> dotprod79/1
  dotprod78/1 -> Mux/78
  "IW{2,1}(78,:)'"/1 -> dotprod78/1
  dotprod77/1 -> Mux/77
  "IW{2,1}(77,:)'"/1 -> dotprod77/1
  dotprod76/1 -> Mux/76
  "IW{2,1}(76,:)'"/1 -> dotprod76/1
  dotprod75/1 -> Mux/75
  "IW{2,1}(75,:)'"/1 -> dotprod75/1
  dotprod74/1 -> Mux/74
  "IW{2,1}(74,:)'"/1 -> dotprod74/1
  dotprod73/1 -> Mux/73
  "IW{2,1}(73,:)'"/1 -> dotprod73/1
  dotprod72/1 -> Mux/72
  "IW{2,1}(72,:)'"/1 -> dotprod72/1
  dotprod71/1 -> Mux/71
  "IW{2,1}(71,:)'"/1 -> dotprod71/1
  dotprod70/1 -> Mux/70
  "IW{2,1}(70,:)'"/1 -> dotprod70/1
  dotprod69/1 -> Mux/69
  "IW{2,1}(69,:)'"/1 -> dotprod69/1
  dotprod68/1 -> Mux/68
  "IW{2,1}(68,:)'"/1 -> dotprod68/1
  dotprod67/1 -> Mux/67
  "IW{2,1}(67,:)'"/1 -> dotprod67/1
  dotprod66/1 -> Mux/66
  "IW{2,1}(66,:)'"/1 -> dotprod66/1
  dotprod65/1 -> Mux/65
  "IW{2,1}(65,:)'"/1 -> dotprod65/1
  dotprod64/1 -> Mux/64
  "IW{2,1}(64,:)'"/1 -> dotprod64/1
  dotprod63/1 -> Mux/63
  "IW{2,1}(63,:)'"/1 -> dotprod63/1
  dotprod62/1 -> Mux/62
  "IW{2,1}(62,:)'"/1 -> dotprod62/1
  dotprod61/1 -> Mux/61
  "IW{2,1}(61,:)'"/1 -> dotprod61/1
  dotprod60/1 -> Mux/60
  "IW{2,1}(60,:)'"/1 -> dotprod60/1
  dotprod59/1 -> Mux/59
  "IW{2,1}(59,:)'"/1 -> dotprod59/1
  dotprod58/1 -> Mux/58
  "IW{2,1}(58,:)'"/1 -> dotprod58/1
  dotprod57/1 -> Mux/57
  "IW{2,1}(57,:)'"/1 -> dotprod57/1
  dotprod56/1 -> Mux/56
  "IW{2,1}(56,:)'"/1 -> dotprod56/1
  dotprod55/1 -> Mux/55
  "IW{2,1}(55,:)'"/1 -> dotprod55/1
  dotprod54/1 -> Mux/54
  "IW{2,1}(54,:)'"/1 -> dotprod54/1
  dotprod53/1 -> Mux/53
  "IW{2,1}(53,:)'"/1 -> dotprod53/1
  dotprod52/1 -> Mux/52
  "IW{2,1}(52,:)'"/1 -> dotprod52/1
  dotprod51/1 -> Mux/51
  "IW{2,1}(51,:)'"/1 -> dotprod51/1
  dotprod50/1 -> Mux/50
  "IW{2,1}(50,:)'"/1 -> dotprod50/1
  dotprod49/1 -> Mux/49
  "IW{2,1}(49,:)'"/1 -> dotprod49/1
  dotprod48/1 -> Mux/48
  "IW{2,1}(48,:)'"/1 -> dotprod48/1
  dotprod47/1 -> Mux/47
  "IW{2,1}(47,:)'"/1 -> dotprod47/1
  dotprod46/1 -> Mux/46
  "IW{2,1}(46,:)'"/1 -> dotprod46/1
  dotprod45/1 -> Mux/45
  "IW{2,1}(45,:)'"/1 -> dotprod45/1
  dotprod44/1 -> Mux/44
  "IW{2,1}(44,:)'"/1 -> dotprod44/1
  dotprod43/1 -> Mux/43
  "IW{2,1}(43,:)'"/1 -> dotprod43/1
  dotprod42/1 -> Mux/42
  "IW{2,1}(42,:)'"/1 -> dotprod42/1
  dotprod41/1 -> Mux/41
  "IW{2,1}(41,:)'"/1 -> dotprod41/1
  dotprod40/1 -> Mux/40
  "IW{2,1}(40,:)'"/1 -> dotprod40/1
  dotprod39/1 -> Mux/39
  "IW{2,1}(39,:)'"/1 -> dotprod39/1
  dotprod38/1 -> Mux/38
  "IW{2,1}(38,:)'"/1 -> dotprod38/1
  dotprod37/1 -> Mux/37
  "IW{2,1}(37,:)'"/1 -> dotprod37/1
  dotprod36/1 -> Mux/36
  "IW{2,1}(36,:)'"/1 -> dotprod36/1
  dotprod35/1 -> Mux/35
  "IW{2,1}(35,:)'"/1 -> dotprod35/1
  dotprod34/1 -> Mux/34
  "IW{2,1}(34,:)'"/1 -> dotprod34/1
  dotprod33/1 -> Mux/33
  "IW{2,1}(33,:)'"/1 -> dotprod33/1
  dotprod32/1 -> Mux/32
  "IW{2,1}(32,:)'"/1 -> dotprod32/1
  dotprod31/1 -> Mux/31
  "IW{2,1}(31,:)'"/1 -> dotprod31/1
  dotprod30/1 -> Mux/30
  "IW{2,1}(30,:)'"/1 -> dotprod30/1
  dotprod29/1 -> Mux/29
  "IW{2,1}(29,:)'"/1 -> dotprod29/1
  dotprod28/1 -> Mux/28
  "IW{2,1}(28,:)'"/1 -> dotprod28/1
  dotprod27/1 -> Mux/27
  "IW{2,1}(27,:)'"/1 -> dotprod27/1
  dotprod26/1 -> Mux/26
  "IW{2,1}(26,:)'"/1 -> dotprod26/1
  dotprod25/1 -> Mux/25
  "IW{2,1}(25,:)'"/1 -> dotprod25/1
  dotprod24/1 -> Mux/24
  "IW{2,1}(24,:)'"/1 -> dotprod24/1
  dotprod23/1 -> Mux/23
  "IW{2,1}(23,:)'"/1 -> dotprod23/1
  dotprod22/1 -> Mux/22
  "IW{2,1}(22,:)'"/1 -> dotprod22/1
  dotprod21/1 -> Mux/21
  "IW{2,1}(21,:)'"/1 -> dotprod21/1
  dotprod20/1 -> Mux/20
  "IW{2,1}(20,:)'"/1 -> dotprod20/1
  dotprod19/1 -> Mux/19
  "IW{2,1}(19,:)'"/1 -> dotprod19/1
  dotprod18/1 -> Mux/18
  "IW{2,1}(18,:)'"/1 -> dotprod18/1
  dotprod17/1 -> Mux/17
  "IW{2,1}(17,:)'"/1 -> dotprod17/1
  dotprod16/1 -> Mux/16
  "IW{2,1}(16,:)'"/1 -> dotprod16/1
  dotprod15/1 -> Mux/15
  "IW{2,1}(15,:)'"/1 -> dotprod15/1
  dotprod14/1 -> Mux/14
  "IW{2,1}(14,:)'"/1 -> dotprod14/1
  dotprod13/1 -> Mux/13
  "IW{2,1}(13,:)'"/1 -> dotprod13/1
  dotprod12/1 -> Mux/12
  "IW{2,1}(12,:)'"/1 -> dotprod12/1
  dotprod11/1 -> Mux/11
  "IW{2,1}(11,:)'"/1 -> dotprod11/1
  dotprod10/1 -> Mux/10
  "IW{2,1}(10,:)'"/1 -> dotprod10/1
  dotprod9/1 -> Mux/9
  "IW{2,1}(9,:)'"/1 -> dotprod9/1
  dotprod8/1 -> Mux/8
  "IW{2,1}(8,:)'"/1 -> dotprod8/1
  dotprod7/1 -> Mux/7
  "IW{2,1}(7,:)'"/1 -> dotprod7/1
  dotprod6/1 -> Mux/6
  "IW{2,1}(6,:)'"/1 -> dotprod6/1
  dotprod5/1 -> Mux/5
  "IW{2,1}(5,:)'"/1 -> dotprod5/1
  dotprod4/1 -> Mux/4
  "IW{2,1}(4,:)'"/1 -> dotprod4/1
  dotprod3/1 -> Mux/3
  "IW{2,1}(3,:)'"/1 -> dotprod3/1
  dotprod2/1 -> Mux/2
  "IW{2,1}(2,:)'"/1 -> dotprod2/1
  dotprod1/1 -> Mux/1
